simulink model "PreCondition"  (R2018b)
settings: Solver=FixedStepDiscrete  StartTime=0.0  StopTime=10.0  FixedStep=0.01  RelTol=1e-3
undefined symbols (not defined in the file or in its folder): EnergyMgLdShdRq1, HMI_2L_StMd10_Config_Val, HMI_2L_StMd11_Config_Val, HMI_2L_StMd12_Config_Val, HMI_2L_StMd13_Config_Val, HMI_2L_StMd14_Config_Val, HMI_2L_StMd15_Config_Val, HMI_2L_StMd16_Config_Val, HMI_2L_StMd17_Config_Val, HMI_2L_StMd18_Config_Val, HMI_2L_StMd19_Config_Val, HMI_2L_StMd1_Config_Val, HMI_2L_StMd20_Config_Val, HMI_2L_StMd21_Config_Val, HMI_2L_StMd22_Config_Val, HMI_2L_StMd23_Config_Val, HMI_2L_StMd24_Config_Val, HMI_2L_StMd25_Config_Val, HMI_2L_StMd26_Config_Val, HMI_2L_StMd27_Config_Val, HMI_2L_StMd28_Config_Val, HMI_2L_StMd29_Config_Val, HMI_2L_StMd2_Config_Val, HMI_2L_StMd30_Config_Val, HMI_2L_StMd31_Config_Val, HMI_2L_StMd32_Config_Val, HMI_2L_StMd3_Config_Val, HMI_2L_StMd4_Config_Val, HMI_2L_StMd5_Config_Val, HMI_2L_StMd6_Config_Val, HMI_2L_StMd7_Config_Val, HMI_2L_StMd8_Config_Val, HMI_2L_StMd9_Config_Val, HMI_2R_StMd10_Config_Val, HMI_2R_StMd11_Config_Val, HMI_2R_StMd12_Config_Val, HMI_2R_StMd13_Config_Val, HMI_2R_StMd14_Config_Val, HMI_2R_StMd15_Config_Val, HMI_2R_StMd16_Config_Val, HMI_2R_StMd17_Config_Val, HMI_2R_StMd18_Config_Val, HMI_2R_StMd19_Config_Val, HMI_2R_StMd1_Config_Val, HMI_2R_StMd20_Config_Val, HMI_2R_StMd21_Config_Val, HMI_2R_StMd22_Config_Val, HMI_2R_StMd23_Config_Val, HMI_2R_StMd24_Config_Val, HMI_2R_StMd25_Config_Val, HMI_2R_StMd26_Config_Val, HMI_2R_StMd27_Config_Val, HMI_2R_StMd28_Config_Val, HMI_2R_StMd29_Config_Val, HMI_2R_StMd2_Config_Val, HMI_2R_StMd30_Config_Val, HMI_2R_StMd31_Config_Val, HMI_2R_StMd32_Config_Val, HMI_2R_StMd3_Config_Val, HMI_2R_StMd4_Config_Val ... (+94)
(part 1 of 6)
settings Model: PauseTimes=0.01  Creator=su3dcu  LastModifiedBy=su3dcu
settings DataIOCC: SaveFormat=StructureWithTime  ReturnWorkspaceOutputs=on
settings OptimizationCC: DefaultParameterBehavior=Inlined  EnhancedBackFolding=on  PassReuseOutputArgsAs=Individual arguments  ZeroExternalMemoryAtStartup=off  ZeroInternalMemoryAtStartup=off  OptimizeBlockOrder=speed  DifferentSizesBufferReuse=on  OptimizationCustomize=off
settings DebuggingCC: ParameterTunabilityLossMsg=error
settings HardwareCC: ProdBitPerPointer=32  ProdBitPerSizeT=32  ProdBitPerPtrDiffT=32  ProdLargestAtomicFloat=None  ProdWordSize=32  ProdHWDeviceType=Renesas->RH850
settings ModelReferenceCC: ModelReferenceNumInstancesAllowed=Single
settings SFSimCC: SimCustomHeaderCode="#include\"Rte_Type.h\""  MATLABDynamicMemAlloc=off
settings RTWCC: SystemTargetFile=autosar.tlc  GenCodeOnly=on  TemplateMakefile=ert_default_tmf  Description=AUTOSAR  GenerateReport=on  IncludeHyperlinkInReport=on  LaunchReport=on  CodeExecutionProfiling=on  GenerateTraceInfo=on  GenerateTraceReport=on  GenerateTraceReportSl=on  GenerateTraceReportSf=on  GenerateTraceReportEml=on  GenerateCodeMetricsReport=on
settings CodeAppCC: ForceParamTrailComments=on  IgnoreCustomStorageClasses=off  MaxIdLength=63  OperatorAnnotations=on  SimulinkDataObjDesc=on  SFDataObjDesc=on  InsertBlockDesc=on
settings STFCustomTargetCC: TargetLangStandard=C99 (ISO)  MultiwordLength=256  ParMdlRefBuildCompliant=on  CompOptLevelCompliant=on  IncludeMdlTerminateFcn=off  CombineOutputUpdateFcns=on  SuppressErrorStatus=on  ERTCustomFileBanners=on  SupportAbsoluteTime=off  PurelyIntegerCode=on  SupportNonFinite=off  SupportComplex=off  SupportContinuousTime=off  SupportNonInlinedSFcns=off  RemoveResetFunc=on  MATLABClassNameForMDSCustomization=Simulink.SoftwareTarget.ERTCustomization  AutosarCompliant=on  UseToolchainInfoCompliant=on  LookupTableObjectStructAxisOrder=2,1,3,4,...  LUTObjectStructOrderEvenSpacing=Size,Table,Breakpoints  SystemTargetFile=autosar.tlc
settings ERTTargetCC: TargetLangStandard=C99 (ISO)  ConcurrentExecutionCompliant=off  IncludeMdlTerminateFcn=off  SuppressErrorStatus=on  SupportAbsoluteTime=off  PurelyIntegerCode=on  SupportNonFinite=off  SupportComplex=off  ModelStepFunctionPrototypeControlCompliant=off  CPPClassGenCompliant=off  AutosarCompliant=on  LookupTableObjectStructAxisOrder=2,1,3,4,...  LUTObjectStructOrderEvenSpacing=Size,Table,Breakpoints  InlinedParameterPlacement=NonHierarchical  ERTCustomFileTemplate=example_file_process.tlc  ERTFilePackagingFormat=Compact
settings ConfigComp: DVTestSuiteOptimization=CombinedObjectives (Nonlinear Extended)  DVDetectActiveLogic=on  DVDetectOutOfBounds=on

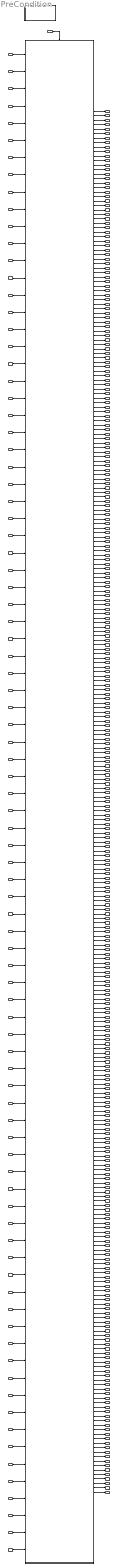
== system PreCondition ==
  PreConitionRunnable : Inport  SampleTime=0.01  OutputFunctionCall=on
  AbgDplyBckp_Val : Inport  Port=2  OutDataTypeStr=boolean  PortDimensions=1
  AbgDplyBckpV_Val : Inport  Port=3  OutDataTypeStr=boolean  PortDimensions=1
  AcsEntryPosLrnd_Val : Inport  Port=4  OutDataTypeStr=PosLrnd1  PortDimensions=1
  DrvStPosRclRspStat_Val : Inport  Port=5  OutDataTypeStr=Enum: PosRclRspStat1  PortDimensions=1
  EnergyMgLdShdRq_Val : Inport  Port=6  OutDataTypeStr=Enum: EnergyMgLdShdRq1  PortDimensions=1
  FamilyLtPosLrnd_Val : Inport  Port=7  OutDataTypeStr=PosLrnd1  PortDimensions=1
  FamilyRtPosLrnd_Val : Inport  Port=8  OutDataTypeStr=PosLrnd1  PortDimensions=1
  IfVeSMSeStNumConfig_Val : Inport  Port=9  OutDataTypeStr=Enum: IfVeSMSeStNumConfig  PortDimensions=1
  IntimacyLPosLrnd_Val : Inport  Port=10  OutDataTypeStr=PosLrnd1  PortDimensions=1
  IntimacyRPosLrnd_Val : Inport  Port=11  OutDataTypeStr=PosLrnd1  PortDimensions=1
  Is2LStSwAct_Val : Inport  Port=12  OutDataTypeStr=boolean  PortDimensions=1
  Is2RStSwAct_Val : Inport  Port=13  OutDataTypeStr=boolean  PortDimensions=1
  Is3LStSwAct_Val : Inport  Port=14  OutDataTypeStr=boolean  PortDimensions=1
  Is3RStSwAct_Val : Inport  Port=15  OutDataTypeStr=boolean  PortDimensions=1
  IsDrvStSwAct_Val : Inport  Port=16  OutDataTypeStr=boolean  PortDimensions=1
  IsPasStSwAct_Val : Inport  Port=17  OutDataTypeStr=boolean  PortDimensions=1
  LgrstCloseLtPosLrnd_Val : Inport  Port=18  OutDataTypeStr=PosLrnd1  PortDimensions=1
  LgrstCloseRtPosLrnd_Val : Inport  Port=19  OutDataTypeStr=PosLrnd1  PortDimensions=1
  LgrstOpenLtPosLrnd_Val : Inport  Port=20  OutDataTypeStr=PosLrnd1  PortDimensions=1
  LgrstOpenRtPosLrnd_Val : Inport  Port=21  OutDataTypeStr=PosLrnd1  PortDimensions=1
  LugLtPosLrnd_Val : Inport  Port=22  OutDataTypeStr=PosLrnd1  PortDimensions=1
  LugRtPosLrnd_Val : Inport  Port=23  OutDataTypeStr=PosLrnd1  PortDimensions=1
  LyingLtPosLrnd_Val : Inport  Port=24  OutDataTypeStr=PosLrnd1  PortDimensions=1
  LyingRtPosLrnd_Val : Inport  Port=25  OutDataTypeStr=PosLrnd1  PortDimensions=1
  MmryRclImpctDisRq_Val : Inport  Port=26  OutDataTypeStr=uint8  PortDimensions=1
  AcsExitPosLrnd_Val : Inport  Port=27  OutDataTypeStr=PosLrnd1  PortDimensions=1
  PassStPosRclRspStat_Val : Inport  Port=28  OutDataTypeStr=Enum: PosRclRspStat1  PortDimensions=1
  VIPLtPosLrnd_Val : Inport  Port=29  OutDataTypeStr=PosLrnd1  PortDimensions=1
  SecRwLtStChldLkReq_Val : Inport  Port=30  OutDataTypeStr=Enum: SeatChldLkSt  PortDimensions=1
  SecRwLtStPosRclRspStat_Val : Inport  Port=31  OutDataTypeStr=Enum: PosRclRspStat1  PortDimensions=1
  VIPRtPosLrnd_Val : Inport  Port=32  OutDataTypeStr=PosLrnd1  PortDimensions=1
  SecRwRtStChldLkReq_Val : Inport  Port=33  OutDataTypeStr=Enum: SeatChldLkSt  PortDimensions=1
  SecRwRtStPosRclRspStat_Val : Inport  Port=34  OutDataTypeStr=Enum: PosRclRspStat1  PortDimensions=1
  SysPwrMd_Val : Inport  Port=35  OutDataTypeStr=Enum: PowerMode1  PortDimensions=1
  SysPwrMdV_Val : Inport  Port=36  OutDataTypeStr=boolean  PortDimensions=1
  ThdRwCtStOccStatMSMSrc_Val : Inport  Port=37  OutDataTypeStr=Enum: SeatOccupiedSts1  PortDimensions=1
  RcvyLtPosLrnd_Val : Inport  Port=38  OutDataTypeStr=PosLrnd1  PortDimensions=1
  ThdRwLtStOccStatMSMSrc_Val : Inport  Port=39  OutDataTypeStr=Enum: SeatOccupiedSts1  PortDimensions=1
  ThdRwLtStPosRclRspStat_Val : Inport  Port=40  OutDataTypeStr=Enum: PosRclRspStat1  PortDimensions=1
  RcvyRtPosLrnd_Val : Inport  Port=41  OutDataTypeStr=PosLrnd1  PortDimensions=1
  ThdRwRtStOccStatMSMSrc_Val : Inport  Port=42  OutDataTypeStr=Enum: SeatOccupiedSts1  PortDimensions=1
  ThdRwRtStPosRclRspStat_Val : Inport  Port=43  OutDataTypeStr=Enum: PosRclRspStat1  PortDimensions=1
  VehMovState_Val : Inport  Port=44  OutDataTypeStr=Enum: VehMovState1  PortDimensions=1
  VehSpdAvgDrvn_Val : Inport  Port=45  OutDataTypeStr=uint16  PortDimensions=1
  VehSpdAvgDrvnV_Val : Inport  Port=46  OutDataTypeStr=boolean  PortDimensions=1
  VeSignalLost2R_463_2L_Val : Inport  Port=47  OutDataTypeStr=boolean  PortDimensions=1
  VeSignalLost3L_468_2L_Val : Inport  Port=48  OutDataTypeStr=boolean  PortDimensions=1
  VeSignalLost3R_46C_2L_Val : Inport  Port=49  OutDataTypeStr=boolean  PortDimensions=1
  VeSignalLostCODR_470_2L_Val : Inport  Port=50  OutDataTypeStr=boolean  PortDimensions=1
  VeSignalLostDR_213_2L_Val : Inport  Port=51  OutDataTypeStr=boolean  PortDimensions=1
  VeSignalLostFireWall_1D2_2L_Val : Inport  Port=52  OutDataTypeStr=boolean  PortDimensions=1
  VeSignalLostSDM_195_2L_Val : Inport  Port=53  OutDataTypeStr=boolean  PortDimensions=1
  VoltSts_Val : Inport  Port=54  OutDataTypeStr=Enum: SeatSysVoltSt  PortDimensions=1
  SecRwLtStFrwdBkwdPos_Val : Inport  Port=55  OutDataTypeStr=uint16  PortDimensions=1
  SecRwLtStFrwdBkwdPosV_Val : Inport  Port=56  OutDataTypeStr=boolean  PortDimensions=1
  SecRwRtStFrwdBkwdPos_Val : Inport  Port=57  OutDataTypeStr=uint16  PortDimensions=1
  SecRwRtStFrwdBkwdPosV_Val : Inport  Port=58  OutDataTypeStr=boolean  PortDimensions=1
  AcsEntry4s2LPosLrnd_Val : Inport  Port=59  OutDataTypeStr=PosLrnd1  PortDimensions=1
  AcsEntry4s2RPosLrnd_Val : Inport  Port=60  OutDataTypeStr=PosLrnd1  PortDimensions=1
  AcsEntryAll4sBwdPosLrnd_Val : Inport  Port=61  OutDataTypeStr=PosLrnd1  PortDimensions=1
  AcsEntryAll4sFwdPosLrnd_Val : Inport  Port=62  OutDataTypeStr=PosLrnd1  PortDimensions=1
  AcsExit4s2LPosLrnd_Val : Inport  Port=63  OutDataTypeStr=PosLrnd1  PortDimensions=1
  AcsExit4s2RPosLrnd_Val : Inport  Port=64  OutDataTypeStr=PosLrnd1  PortDimensions=1
  IfVeSMSbPassReclinerPosLrnd_Val : Inport  Port=65  OutDataTypeStr=PosLrnd1  PortDimensions=1
  IfVeSMSbunfold3LPosLrnd_Val : Inport  Port=66  OutDataTypeStr=PosLrnd1  PortDimensions=1
  IfVeSMSbunfold3RPosLrnd_Val : Inport  Port=67  OutDataTypeStr=PosLrnd1  PortDimensions=1
  NotCoDrvStOccStatBDFSrc_Val : Inport  Port=68  OutDataTypeStr=Enum: SeatOccupiedSts1  PortDimensions=1
  IfVeSMSbVIPLtOutPosLrnd_Val : Inport  Port=69  OutDataTypeStr=PosLrnd1  PortDimensions=1
  IfVeSMSbVIPRtOutPosLrnd_Val : Inport  Port=70  OutDataTypeStr=PosLrnd1  PortDimensions=1
  IfVeSMSuThdRwLtStCshnFldUpwdDnwdPos_Val : Inport  Port=71  OutDataTypeStr=uint16  PortDimensions=1
  IfVeSMSuThdRwLtStCshnFldUpwdDnwdPosV_Val : Inport  Port=72  OutDataTypeStr=boolean  PortDimensions=1
  IfVeSMSuThdRwRtStCshnFldUpwdDnwdPos_Val : Inport  Port=73  OutDataTypeStr=uint16  PortDimensions=1
  IfVeSMSuThdRwRtStCshnFldUpwdDnwdPosV_Val : Inport  Port=74  OutDataTypeStr=boolean  PortDimensions=1
  ThdRwLtStChldLkReq_Val : Inport  Port=75  OutDataTypeStr=Enum: SeatChldLkSt  PortDimensions=1
  NotSecRowLeStOccStatBDFSrc_Val : Inport  Port=76  OutDataTypeStr=Enum: SeatOccupiedSts1  PortDimensions=1
  NotSecRowRtStOccStatBDFSrc_Val : Inport  Port=77  OutDataTypeStr=Enum: SeatOccupiedSts1  PortDimensions=1
  IfVeSMSbSecRwLtStBkReclnUpwdDnwdPosV_Val : Inport  Port=78  OutDataTypeStr=boolean  PortDimensions=1
  IfVeSMSbSecRwRtStBkReclnUpwdDnwdPosV_Val : Inport  Port=79  OutDataTypeStr=boolean  PortDimensions=1
  IfVeSMSuSecRwLtStBkReclnUpwdDnwdPos_Val : Inport  Port=80  OutDataTypeStr=uint16  PortDimensions=1
  IfVeSMSuSecRwRtStBkReclnUpwdDnwdPos_Val : Inport  Port=81  OutDataTypeStr=uint16  PortDimensions=1
  IfVeSMSbPasReclinerPosAvail_Val : Inport  Port=82  OutDataTypeStr=boolean  PortDimensions=1
  WholeVehMemPosLrnd_Val : Inport  Port=83  OutDataTypeStr=PosLrnd1  PortDimensions=1
  Md61PassStBkReclnTrgtPos_Val : Inport  Port=84  OutDataTypeStr=uint16  PortDimensions=1
  Md61ThdRwLtStCshnFldUpwdDnwdTrgtPos_Val : Inport  Port=85  OutDataTypeStr=uint16  PortDimensions=1
  Md61ThdRwRtStCshnFldUpwdDnwdTrgtPos_Val : Inport  Port=86  OutDataTypeStr=uint16  PortDimensions=1
  Md62PassStBkReclnTrgtPos_Val : Inport  Port=87  OutDataTypeStr=uint16  PortDimensions=1
  Md62ThdRwLtStCshnFldUpwdDnwdTrgtPos_Val : Inport  Port=88  OutDataTypeStr=uint16  PortDimensions=1
  Md62ThdRwRtStCshnFldUpwdDnwdTrgtPos_Val : Inport  Port=89  OutDataTypeStr=uint16  PortDimensions=1
  PreCondition_Init : Subsystem
  PreConitionRunnable_sys : Subsystem
  AcsMdEntyAvl_Val : Outport  OutDataTypeStr=boolean  PortDimensions=1
  AcsMdExtAvl_Val : Outport  Port=2  OutDataTypeStr=boolean  PortDimensions=1
  CommCond_Val : Outport  Port=3  OutDataTypeStr=boolean  PortDimensions=1
  CommExitCond_Val : Outport  Port=4  OutDataTypeStr=boolean  PortDimensions=1
  CommExitCondwithSpeed_Val : Outport  Port=5  OutDataTypeStr=boolean  PortDimensions=1
  DiagAbgDly_Val : Outport  Port=6  OutDataTypeStr=Enum: DiagAbgDly  PortDimensions=1
  DiagVehMovState_Val : Outport  Port=7  OutDataTypeStr=Enum: DiagVehMovState  PortDimensions=1
  DiagVehSpdAvgDrvn_Val : Outport  Port=8  OutDataTypeStr=Enum: DiagVehSpdAvgDrvn  PortDimensions=1
  FamilyMdLtAvl_Val : Outport  Port=9  OutDataTypeStr=boolean  PortDimensions=1
  FamilyMdRtAvl_Val : Outport  Port=10  OutDataTypeStr=boolean  PortDimensions=1
  HMIMd10Avl_2L_Val : Outport  Port=11  OutDataTypeStr=boolean  PortDimensions=1
  HMIMd10Avl_2R_Val : Outport  Port=12  OutDataTypeStr=boolean  PortDimensions=1
  HMIMd10Cfg_2L_Val : Outport  Port=13  OutDataTypeStr=boolean  PortDimensions=1
  HMIMd10Cfg_2R_Val : Outport  Port=14  OutDataTypeStr=boolean  PortDimensions=1
  HMIMd11Avl_2L_Val : Outport  Port=15  OutDataTypeStr=boolean  PortDimensions=1
  HMIMd11Avl_2R_Val : Outport  Port=16  OutDataTypeStr=boolean  PortDimensions=1
  HMIMd11Cfg_2L_Val : Outport  Port=17  OutDataTypeStr=boolean  PortDimensions=1
  HMIMd11Cfg_2R_Val : Outport  Port=18  OutDataTypeStr=boolean  PortDimensions=1
  HMIMd12Avl_2L_Val : Outport  Port=19  OutDataTypeStr=boolean  PortDimensions=1
  HMIMd12Avl_2R_Val : Outport  Port=20  OutDataTypeStr=boolean  PortDimensions=1
  HMIMd12Cfg_2L_Val : Outport  Port=21  OutDataTypeStr=boolean  PortDimensions=1
  HMIMd12Cfg_2R_Val : Outport  Port=22  OutDataTypeStr=boolean  PortDimensions=1
  HMIMd13Avl_2L_Val : Outport  Port=23  OutDataTypeStr=boolean  PortDimensions=1
  HMIMd13Avl_2R_Val : Outport  Port=24  OutDataTypeStr=boolean  PortDimensions=1
  HMIMd13Cfg_2L_Val : Outport  Port=25  OutDataTypeStr=boolean  PortDimensions=1
  HMIMd13Cfg_2R_Val : Outport  Port=26  OutDataTypeStr=boolean  PortDimensions=1
  HMIMd14Avl_2L_Val : Outport  Port=27  OutDataTypeStr=boolean  PortDimensions=1
  HMIMd14Avl_2R_Val : Outport  Port=28  OutDataTypeStr=boolean  PortDimensions=1
  HMIMd14Cfg_2L_Val : Outport  Port=29  OutDataTypeStr=boolean  PortDimensions=1
  HMIMd14Cfg_2R_Val : Outport  Port=30  OutDataTypeStr=boolean  PortDimensions=1
  HMIMd15Avl_2L_Val : Outport  Port=31  OutDataTypeStr=boolean  PortDimensions=1
  HMIMd15Avl_2R_Val : Outport  Port=32  OutDataTypeStr=boolean  PortDimensions=1
  HMIMd15Cfg_2L_Val : Outport  Port=33  OutDataTypeStr=boolean  PortDimensions=1
  HMIMd15Cfg_2R_Val : Outport  Port=34  OutDataTypeStr=boolean  PortDimensions=1
  HMIMd16Avl_2L_Val : Outport  Port=35  OutDataTypeStr=boolean  PortDimensions=1
  HMIMd16Avl_2R_Val : Outport  Port=36  OutDataTypeStr=boolean  PortDimensions=1
  HMIMd16Cfg_2L_Val : Outport  Port=37  OutDataTypeStr=boolean  PortDimensions=1
  HMIMd16Cfg_2R_Val : Outport  Port=38  OutDataTypeStr=boolean  PortDimensions=1
  HMIMd17Avl_2L_Val : Outport  Port=39  OutDataTypeStr=boolean  PortDimensions=1
  HMIMd17Avl_2R_Val : Outport  Port=40  OutDataTypeStr=boolean  PortDimensions=1
  HMIMd17Cfg_2L_Val : Outport  Port=41  OutDataTypeStr=boolean  PortDimensions=1
  HMIMd17Cfg_2R_Val : Outport  Port=42  OutDataTypeStr=boolean  PortDimensions=1
  HMIMd18Avl_2L_Val : Outport  Port=43  OutDataTypeStr=boolean  PortDimensions=1
  HMIMd18Avl_2R_Val : Outport  Port=44  OutDataTypeStr=boolean  PortDimensions=1
  HMIMd18Cfg_2L_Val : Outport  Port=45  OutDataTypeStr=boolean  PortDimensions=1
  HMIMd18Cfg_2R_Val : Outport  Port=46  OutDataTypeStr=boolean  PortDimensions=1
  HMIMd19Avl_2L_Val : Outport  Port=47  OutDataTypeStr=boolean  PortDimensions=1
  HMIMd19Avl_2R_Val : Outport  Port=48  OutDataTypeStr=boolean  PortDimensions=1
  HMIMd19Cfg_2L_Val : Outport  Port=49  OutDataTypeStr=boolean  PortDimensions=1
  HMIMd19Cfg_2R_Val : Outport  Port=50  OutDataTypeStr=boolean  PortDimensions=1
  HMIMd1Avl_2L_Val : Outport  Port=51  OutDataTypeStr=boolean  PortDimensions=1
  HMIMd1Avl_2R_Val : Outport  Port=52  OutDataTypeStr=boolean  PortDimensions=1
  HMIMd1Cfg_2L_Val : Outport  Port=53  OutDataTypeStr=boolean  PortDimensions=1
  HMIMd1Cfg_2R_Val : Outport  Port=54  OutDataTypeStr=boolean  PortDimensions=1
  HMIMd20Avl_2L_Val : Outport  Port=55  OutDataTypeStr=boolean  PortDimensions=1
  HMIMd20Avl_2R_Val : Outport  Port=56  OutDataTypeStr=boolean  PortDimensions=1
  HMIMd20Cfg_2L_Val : Outport  Port=57  OutDataTypeStr=boolean  PortDimensions=1
  HMIMd20Cfg_2R_Val : Outport  Port=58  OutDataTypeStr=boolean  PortDimensions=1
  HMIMd21Avl_2L_Val : Outport  Port=59  OutDataTypeStr=boolean  PortDimensions=1
  HMIMd21Avl_2R_Val : Outport  Port=60  OutDataTypeStr=boolean  PortDimensions=1
  HMIMd21Cfg_2L_Val : Outport  Port=61  OutDataTypeStr=boolean  PortDimensions=1
  HMIMd21Cfg_2R_Val : Outport  Port=62  OutDataTypeStr=boolean  PortDimensions=1
  HMIMd22Avl_2L_Val : Outport  Port=63  OutDataTypeStr=boolean  PortDimensions=1
  HMIMd22Avl_2R_Val : Outport  Port=64  OutDataTypeStr=boolean  PortDimensions=1
  HMIMd22Cfg_2L_Val : Outport  Port=65  OutDataTypeStr=boolean  PortDimensions=1
  HMIMd22Cfg_2R_Val : Outport  Port=66  OutDataTypeStr=boolean  PortDimensions=1
  HMIMd23Avl_2L_Val : Outport  Port=67  OutDataTypeStr=boolean  PortDimensions=1
  HMIMd23Avl_2R_Val : Outport  Port=68  OutDataTypeStr=boolean  PortDimensions=1
  HMIMd23Cfg_2L_Val : Outport  Port=69  OutDataTypeStr=boolean  PortDimensions=1
  HMIMd23Cfg_2R_Val : Outport  Port=70  OutDataTypeStr=boolean  PortDimensions=1
  HMIMd24Avl_2L_Val : Outport  Port=71  OutDataTypeStr=boolean  PortDimensions=1
  HMIMd24Avl_2R_Val : Outport  Port=72  OutDataTypeStr=boolean  PortDimensions=1
  HMIMd24Cfg_2L_Val : Outport  Port=73  OutDataTypeStr=boolean  PortDimensions=1
  HMIMd24Cfg_2R_Val : Outport  Port=74  OutDataTypeStr=boolean  PortDimensions=1
  HMIMd25Avl_2L_Val : Outport  Port=75  OutDataTypeStr=boolean  PortDimensions=1
  HMIMd25Avl_2R_Val : Outport  Port=76  OutDataTypeStr=boolean  PortDimensions=1
  HMIMd25Cfg_2L_Val : Outport  Port=77  OutDataTypeStr=boolean  PortDimensions=1
  HMIMd25Cfg_2R_Val : Outport  Port=78  OutDataTypeStr=boolean  PortDimensions=1
  HMIMd26Avl_2L_Val : Outport  Port=79  OutDataTypeStr=boolean  PortDimensions=1
  HMIMd26Avl_2R_Val : Outport  Port=80  OutDataTypeStr=boolean  PortDimensions=1
  HMIMd26Cfg_2L_Val : Outport  Port=81  OutDataTypeStr=boolean  PortDimensions=1
  HMIMd26Cfg_2R_Val : Outport  Port=82  OutDataTypeStr=boolean  PortDimensions=1
  HMIMd27Avl_2L_Val : Outport  Port=83  OutDataTypeStr=boolean  PortDimensions=1
  HMIMd27Avl_2R_Val : Outport  Port=84  OutDataTypeStr=boolean  PortDimensions=1
  HMIMd27Cfg_2L_Val : Outport  Port=85  OutDataTypeStr=boolean  PortDimensions=1
  HMIMd27Cfg_2R_Val : Outport  Port=86  OutDataTypeStr=boolean  PortDimensions=1
  HMIMd28Avl_2L_Val : Outport  Port=87  OutDataTypeStr=boolean  PortDimensions=1
  HMIMd28Avl_2R_Val : Outport  Port=88  OutDataTypeStr=boolean  PortDimensions=1
  HMIMd28Cfg_2L_Val : Outport  Port=89  OutDataTypeStr=boolean  PortDimensions=1
  HMIMd28Cfg_2R_Val : Outport  Port=90  OutDataTypeStr=boolean  PortDimensions=1
  HMIMd29Avl_2L_Val : Outport  Port=91  OutDataTypeStr=boolean  PortDimensions=1
  HMIMd29Avl_2R_Val : Outport  Port=92  OutDataTypeStr=boolean  PortDimensions=1
  HMIMd29Cfg_2L_Val : Outport  Port=93  OutDataTypeStr=boolean  PortDimensions=1
  HMIMd29Cfg_2R_Val : Outport  Port=94  OutDataTypeStr=boolean  PortDimensions=1
  HMIMd2Avl_2L_Val : Outport  Port=95  OutDataTypeStr=boolean  PortDimensions=1
  HMIMd2Avl_2R_Val : Outport  Port=96  OutDataTypeStr=boolean  PortDimensions=1
  HMIMd2Cfg_2L_Val : Outport  Port=97  OutDataTypeStr=boolean  PortDimensions=1
  HMIMd2Cfg_2R_Val : Outport  Port=98  OutDataTypeStr=boolean  PortDimensions=1
  HMIMd30Avl_2L_Val : Outport  Port=99  OutDataTypeStr=boolean  PortDimensions=1
  HMIMd30Avl_2R_Val : Outport  Port=100  OutDataTypeStr=boolean  PortDimensions=1
  HMIMd30Cfg_2L_Val : Outport  Port=101  OutDataTypeStr=boolean  PortDimensions=1
  HMIMd30Cfg_2R_Val : Outport  Port=102  OutDataTypeStr=boolean  PortDimensions=1
  HMIMd31Avl_2L_Val : Outport  Port=103  OutDataTypeStr=boolean  PortDimensions=1
  HMIMd31Avl_2R_Val : Outport  Port=104  OutDataTypeStr=boolean  PortDimensions=1
  HMIMd31Cfg_2L_Val : Outport  Port=105  OutDataTypeStr=boolean  PortDimensions=1
  HMIMd31Cfg_2R_Val : Outport  Port=106  OutDataTypeStr=boolean  PortDimensions=1
  HMIMd32Avl_2L_Val : Outport  Port=107  OutDataTypeStr=boolean  PortDimensions=1
  HMIMd32Avl_2R_Val : Outport  Port=108  OutDataTypeStr=boolean  PortDimensions=1
  HMIMd32Cfg_2L_Val : Outport  Port=109  OutDataTypeStr=boolean  PortDimensions=1
  HMIMd32Cfg_2R_Val : Outport  Port=110  OutDataTypeStr=boolean  PortDimensions=1
  HMIMd3Avl_2L_Val : Outport  Port=111  OutDataTypeStr=boolean  PortDimensions=1
  HMIMd3Avl_2R_Val : Outport  Port=112  OutDataTypeStr=boolean  PortDimensions=1
  HMIMd3Cfg_2L_Val : Outport  Port=113  OutDataTypeStr=boolean  PortDimensions=1
  HMIMd3Cfg_2R_Val : Outport  Port=114  OutDataTypeStr=boolean  PortDimensions=1
  HMIMd4Avl_2L_Val : Outport  Port=115  OutDataTypeStr=boolean  PortDimensions=1
  HMIMd4Avl_2R_Val : Outport  Port=116  OutDataTypeStr=boolean  PortDimensions=1
  HMIMd4Cfg_2L_Val : Outport  Port=117  OutDataTypeStr=boolean  PortDimensions=1
  HMIMd4Cfg_2R_Val : Outport  Port=118  OutDataTypeStr=boolean  PortDimensions=1
  HMIMd5Avl_2L_Val : Outport  Port=119  OutDataTypeStr=boolean  PortDimensions=1
  HMIMd5Avl_2R_Val : Outport  Port=120  OutDataTypeStr=boolean  PortDimensions=1
  HMIMd5Cfg_2L_Val : Outport  Port=121  OutDataTypeStr=boolean  PortDimensions=1
  HMIMd5Cfg_2R_Val : Outport  Port=122  OutDataTypeStr=boolean  PortDimensions=1
  HMIMd6Avl_2L_Val : Outport  Port=123  OutDataTypeStr=boolean  PortDimensions=1
  HMIMd6Avl_2R_Val : Outport  Port=124  OutDataTypeStr=boolean  PortDimensions=1
  HMIMd6Cfg_2L_Val : Outport  Port=125  OutDataTypeStr=boolean  PortDimensions=1
  HMIMd6Cfg_2R_Val : Outport  Port=126  OutDataTypeStr=boolean  PortDimensions=1
  HMIMd7Avl_2L_Val : Outport  Port=127  OutDataTypeStr=boolean  PortDimensions=1
  HMIMd7Avl_2R_Val : Outport  Port=128  OutDataTypeStr=boolean  PortDimensions=1
  HMIMd7Cfg_2L_Val : Outport  Port=129  OutDataTypeStr=boolean  PortDimensions=1
  HMIMd7Cfg_2R_Val : Outport  Port=130  OutDataTypeStr=boolean  PortDimensions=1
  HMIMd8Avl_2L_Val : Outport  Port=131  OutDataTypeStr=boolean  PortDimensions=1
  HMIMd8Avl_2R_Val : Outport  Port=132  OutDataTypeStr=boolean  PortDimensions=1
  HMIMd8Cfg_2L_Val : Outport  Port=133  OutDataTypeStr=boolean  PortDimensions=1
  HMIMd8Cfg_2R_Val : Outport  Port=134  OutDataTypeStr=boolean  PortDimensions=1
  HMIMd9Avl_2L_Val : Outport  Port=135  OutDataTypeStr=boolean  PortDimensions=1
  HMIMd9Avl_2R_Val : Outport  Port=136  OutDataTypeStr=boolean  PortDimensions=1
  HMIMd9Cfg_2L_Val : Outport  Port=137  OutDataTypeStr=boolean  PortDimensions=1
  HMIMd9Cfg_2R_Val : Outport  Port=138  OutDataTypeStr=boolean  PortDimensions=1
  IntimacyLMdAvl_Val : Outport  Port=139  OutDataTypeStr=boolean  PortDimensions=1
  IntimacyRMdAvl_Val : Outport  Port=140  OutDataTypeStr=boolean  PortDimensions=1
  LgrstCloseLtMdAvl_Val : Outport  Port=141  OutDataTypeStr=boolean  PortDimensions=1
  LgrstCloseRtMdAvl_Val : Outport  Port=142  OutDataTypeStr=boolean  PortDimensions=1
  LgrstOpenLtMdAvl_Val : Outport  Port=143  OutDataTypeStr=boolean  PortDimensions=1
  LgrstOpenRtMdAvl_Val : Outport  Port=144  OutDataTypeStr=boolean  PortDimensions=1
  LugMdLtAvl_Val : Outport  Port=145  OutDataTypeStr=boolean  PortDimensions=1
  LugMdRtAvl_Val : Outport  Port=146  OutDataTypeStr=boolean  PortDimensions=1
  LyingMdLtAvl_Val : Outport  Port=147  OutDataTypeStr=boolean  PortDimensions=1
  LyingMdRtAvl_Val : Outport  Port=148  OutDataTypeStr=boolean  PortDimensions=1
  PwrMdChked_Val : Outport  Port=149  OutDataTypeStr=Enum: PowerMode1  PortDimensions=1
  RcvyMdLtAvl_Val : Outport  Port=150  OutDataTypeStr=boolean  PortDimensions=1
  RcvyMdRtAvl_Val : Outport  Port=151  OutDataTypeStr=boolean  PortDimensions=1
  StPassCmprtMdCtrl_Md1_VCUAvl_Val : Outport  Port=152  OutDataTypeStr=boolean  PortDimensions=1
  StPassCmprtMdCtrl_Md1_VCUCfg_Val : Outport  Port=153  OutDataTypeStr=boolean  PortDimensions=1
  StPassCmprtMdCtrl_Md10_VCUAvl_Val : Outport  Port=154  OutDataTypeStr=boolean  PortDimensions=1
  StPassCmprtMdCtrl_Md10_VCUCfg_Val : Outport  Port=155  OutDataTypeStr=boolean  PortDimensions=1
  StPassCmprtMdCtrl_Md11_VCUAvl_Val : Outport  Port=156  OutDataTypeStr=boolean  PortDimensions=1
  StPassCmprtMdCtrl_Md11_VCUCfg_Val : Outport  Port=157  OutDataTypeStr=boolean  PortDimensions=1
  StPassCmprtMdCtrl_Md12_VCUAvl_Val : Outport  Port=158  OutDataTypeStr=boolean  PortDimensions=1
  StPassCmprtMdCtrl_Md12_VCUCfg_Val : Outport  Port=159  OutDataTypeStr=boolean  PortDimensions=1
  StPassCmprtMdCtrl_Md13_VCUAvl_Val : Outport  Port=160  OutDataTypeStr=boolean  PortDimensions=1
  StPassCmprtMdCtrl_Md13_VCUCfg_Val : Outport  Port=161  OutDataTypeStr=boolean  PortDimensions=1
  StPassCmprtMdCtrl_Md14_VCUAvl_Val : Outport  Port=162  OutDataTypeStr=boolean  PortDimensions=1
  StPassCmprtMdCtrl_Md14_VCUCfg_Val : Outport  Port=163  OutDataTypeStr=boolean  PortDimensions=1
  StPassCmprtMdCtrl_Md15_VCUAvl_Val : Outport  Port=164  OutDataTypeStr=boolean  PortDimensions=1
  StPassCmprtMdCtrl_Md15_VCUCfg_Val : Outport  Port=165  OutDataTypeStr=boolean  PortDimensions=1
  StPassCmprtMdCtrl_Md16_VCUAvl_Val : Outport  Port=166  OutDataTypeStr=boolean  PortDimensions=1
  StPassCmprtMdCtrl_Md16_VCUCfg_Val : Outport  Port=167  OutDataTypeStr=boolean  PortDimensions=1
  StPassCmprtMdCtrl_Md17_VCUAvl_Val : Outport  Port=168  OutDataTypeStr=boolean  PortDimensions=1
  StPassCmprtMdCtrl_Md17_VCUCfg_Val : Outport  Port=169  OutDataTypeStr=boolean  PortDimensions=1
  StPassCmprtMdCtrl_Md18_VCUAvl_Val : Outport  Port=170  OutDataTypeStr=boolean  PortDimensions=1
  StPassCmprtMdCtrl_Md18_VCUCfg_Val : Outport  Port=171  OutDataTypeStr=boolean  PortDimensions=1
  StPassCmprtMdCtrl_Md19_VCUAvl_Val : Outport  Port=172  OutDataTypeStr=boolean  PortDimensions=1
  StPassCmprtMdCtrl_Md19_VCUCfg_Val : Outport  Port=173  OutDataTypeStr=boolean  PortDimensions=1
  StPassCmprtMdCtrl_Md2_VCUAvl_Val : Outport  Port=174  OutDataTypeStr=boolean  PortDimensions=1
  StPassCmprtMdCtrl_Md2_VCUCfg_Val : Outport  Port=175  OutDataTypeStr=boolean  PortDimensions=1
  StPassCmprtMdCtrl_Md20_VCUAvl_Val : Outport  Port=176  OutDataTypeStr=boolean  PortDimensions=1
  StPassCmprtMdCtrl_Md20_VCUCfg_Val : Outport  Port=177  OutDataTypeStr=boolean  PortDimensions=1
  StPassCmprtMdCtrl_Md21_VCUAvl_Val : Outport  Port=178  OutDataTypeStr=boolean  PortDimensions=1
  StPassCmprtMdCtrl_Md21_VCUCfg_Val : Outport  Port=179  OutDataTypeStr=boolean  PortDimensions=1
  StPassCmprtMdCtrl_Md22_VCUAvl_Val : Outport  Port=180  OutDataTypeStr=boolean  PortDimensions=1
  StPassCmprtMdCtrl_Md22_VCUCfg_Val : Outport  Port=181  OutDataTypeStr=boolean  PortDimensions=1
  StPassCmprtMdCtrl_Md23_VCUAvl_Val : Outport  Port=182  OutDataTypeStr=boolean  PortDimensions=1
  StPassCmprtMdCtrl_Md23_VCUCfg_Val : Outport  Port=183  OutDataTypeStr=boolean  PortDimensions=1
  StPassCmprtMdCtrl_Md24_VCUAvl_Val : Outport  Port=184  OutDataTypeStr=boolean  PortDimensions=1
  StPassCmprtMdCtrl_Md24_VCUCfg_Val : Outport  Port=185  OutDataTypeStr=boolean  PortDimensions=1
  StPassCmprtMdCtrl_Md25_VCUAvl_Val : Outport  Port=186  OutDataTypeStr=boolean  PortDimensions=1
  StPassCmprtMdCtrl_Md25_VCUCfg_Val : Outport  Port=187  OutDataTypeStr=boolean  PortDimensions=1
  StPassCmprtMdCtrl_Md26_VCUAvl_Val : Outport  Port=188  OutDataTypeStr=boolean  PortDimensions=1
  StPassCmprtMdCtrl_Md26_VCUCfg_Val : Outport  Port=189  OutDataTypeStr=boolean  PortDimensions=1
  StPassCmprtMdCtrl_Md27_VCUAvl_Val : Outport  Port=190  OutDataTypeStr=boolean  PortDimensions=1
  StPassCmprtMdCtrl_Md27_VCUCfg_Val : Outport  Port=191  OutDataTypeStr=boolean  PortDimensions=1
  StPassCmprtMdCtrl_Md28_VCUAvl_Val : Outport  Port=192  OutDataTypeStr=boolean  PortDimensions=1
  StPassCmprtMdCtrl_Md28_VCUCfg_Val : Outport  Port=193  OutDataTypeStr=boolean  PortDimensions=1
  StPassCmprtMdCtrl_Md29_VCUAvl_Val : Outport  Port=194  OutDataTypeStr=boolean  PortDimensions=1
  StPassCmprtMdCtrl_Md29_VCUCfg_Val : Outport  Port=195  OutDataTypeStr=boolean  PortDimensions=1
  StPassCmprtMdCtrl_Md3_VCUAvl_Val : Outport  Port=196  OutDataTypeStr=boolean  PortDimensions=1
  StPassCmprtMdCtrl_Md3_VCUCfg_Val : Outport  Port=197  OutDataTypeStr=boolean  PortDimensions=1
  StPassCmprtMdCtrl_Md30_VCUAvl_Val : Outport  Port=198  OutDataTypeStr=boolean  PortDimensions=1
  StPassCmprtMdCtrl_Md30_VCUCfg_Val : Outport  Port=199  OutDataTypeStr=boolean  PortDimensions=1
  StPassCmprtMdCtrl_Md31_VCUAvl_Val : Outport  Port=200  OutDataTypeStr=boolean  PortDimensions=1
  StPassCmprtMdCtrl_Md31_VCUCfg_Val : Outport  Port=201  OutDataTypeStr=boolean  PortDimensions=1
  StPassCmprtMdCtrl_Md32_VCUAvl_Val : Outport  Port=202  OutDataTypeStr=boolean  PortDimensions=1
  StPassCmprtMdCtrl_Md32_VCUCfg_Val : Outport  Port=203  OutDataTypeStr=boolean  PortDimensions=1
  StPassCmprtMdCtrl_Md4_VCUAvl_Val : Outport  Port=204  OutDataTypeStr=boolean  PortDimensions=1
  StPassCmprtMdCtrl_Md4_VCUCfg_Val : Outport  Port=205  OutDataTypeStr=boolean  PortDimensions=1
  StPassCmprtMdCtrl_Md5_VCUAvl_Val : Outport  Port=206  OutDataTypeStr=boolean  PortDimensions=1
  StPassCmprtMdCtrl_Md5_VCUCfg_Val : Outport  Port=207  OutDataTypeStr=boolean  PortDimensions=1
  StPassCmprtMdCtrl_Md6_VCUAvl_Val : Outport  Port=208  OutDataTypeStr=boolean  PortDimensions=1
  StPassCmprtMdCtrl_Md6_VCUCfg_Val : Outport  Port=209  OutDataTypeStr=boolean  PortDimensions=1
  StPassCmprtMdCtrl_Md7_VCUAvl_Val : Outport  Port=210  OutDataTypeStr=boolean  PortDimensions=1
  StPassCmprtMdCtrl_Md7_VCUCfg_Val : Outport  Port=211  OutDataTypeStr=boolean  PortDimensions=1
  StPassCmprtMdCtrl_Md8_VCUAvl_Val : Outport  Port=212  OutDataTypeStr=boolean  PortDimensions=1
  StPassCmprtMdCtrl_Md8_VCUCfg_Val : Outport  Port=213  OutDataTypeStr=boolean  PortDimensions=1
  StPassCmprtMdCtrl_Md9_VCUAvl_Val : Outport  Port=214  OutDataTypeStr=boolean  PortDimensions=1
  StPassCmprtMdCtrl_Md9_VCUCfg_Val : Outport  Port=215  OutDataTypeStr=boolean  PortDimensions=1
  StPassCmprtMdRfCtrlSwCstStAvl_Val : Outport  Port=216  OutDataTypeStr=boolean  PortDimensions=1
  StSrvAvl_Md1_Val : Outport  Port=217  OutDataTypeStr=boolean  PortDimensions=1
  StSrvAvl_Md10_Val : Outport  Port=218  OutDataTypeStr=boolean  PortDimensions=1
  StSrvAvl_Md11_Val : Outport  Port=219  OutDataTypeStr=boolean  PortDimensions=1
  StSrvAvl_Md12_Val : Outport  Port=220  OutDataTypeStr=boolean  PortDimensions=1
  StSrvAvl_Md13_Val : Outport  Port=221  OutDataTypeStr=boolean  PortDimensions=1
  StSrvAvl_Md14_Val : Outport  Port=222  OutDataTypeStr=boolean  PortDimensions=1
  StSrvAvl_Md15_Val : Outport  Port=223  OutDataTypeStr=boolean  PortDimensions=1
  StSrvAvl_Md16_Val : Outport  Port=224  OutDataTypeStr=boolean  PortDimensions=1
  StSrvAvl_Md17_Val : Outport  Port=225  OutDataTypeStr=boolean  PortDimensions=1
  StSrvAvl_Md18_Val : Outport  Port=226  OutDataTypeStr=boolean  PortDimensions=1
  StSrvAvl_Md19_Val : Outport  Port=227  OutDataTypeStr=boolean  PortDimensions=1
  StSrvAvl_Md2_Val : Outport  Port=228  OutDataTypeStr=boolean  PortDimensions=1
  StSrvAvl_Md20_Val : Outport  Port=229  OutDataTypeStr=boolean  PortDimensions=1
  StSrvAvl_Md21_Val : Outport  Port=230  OutDataTypeStr=boolean  PortDimensions=1
  StSrvAvl_Md22_Val : Outport  Port=231  OutDataTypeStr=boolean  PortDimensions=1
  StSrvAvl_Md23_Val : Outport  Port=232  OutDataTypeStr=boolean  PortDimensions=1
  StSrvAvl_Md24_Val : Outport  Port=233  OutDataTypeStr=boolean  PortDimensions=1
  StSrvAvl_Md25_Val : Outport  Port=234  OutDataTypeStr=boolean  PortDimensions=1
  StSrvAvl_Md26_Val : Outport  Port=235  OutDataTypeStr=boolean  PortDimensions=1
  StSrvAvl_Md27_Val : Outport  Port=236  OutDataTypeStr=boolean  PortDimensions=1
  StSrvAvl_Md28_Val : Outport  Port=237  OutDataTypeStr=boolean  PortDimensions=1
  StSrvAvl_Md29_Val : Outport  Port=238  OutDataTypeStr=boolean  PortDimensions=1
  StSrvAvl_Md3_Val : Outport  Port=239  OutDataTypeStr=boolean  PortDimensions=1
  StSrvAvl_Md30_Val : Outport  Port=240  OutDataTypeStr=boolean  PortDimensions=1
  StSrvAvl_Md31_Val : Outport  Port=241  OutDataTypeStr=boolean  PortDimensions=1
  StSrvAvl_Md32_Val : Outport  Port=242  OutDataTypeStr=boolean  PortDimensions=1
  StSrvAvl_Md4_Val : Outport  Port=243  OutDataTypeStr=boolean  PortDimensions=1
  StSrvAvl_Md5_Val : Outport  Port=244  OutDataTypeStr=boolean  PortDimensions=1
  StSrvAvl_Md6_Val : Outport  Port=245  OutDataTypeStr=boolean  PortDimensions=1
  StSrvAvl_Md7_Val : Outport  Port=246  OutDataTypeStr=boolean  PortDimensions=1
  StSrvAvl_Md8_Val : Outport  Port=247  OutDataTypeStr=boolean  PortDimensions=1
  StSrvAvl_Md9_Val : Outport  Port=248  OutDataTypeStr=boolean  PortDimensions=1
  StSrvCfg_Md1_Val : Outport  Port=249  OutDataTypeStr=boolean  PortDimensions=1
  StSrvCfg_Md10_Val : Outport  Port=250  OutDataTypeStr=boolean  PortDimensions=1
  StSrvCfg_Md11_Val : Outport  Port=251  OutDataTypeStr=boolean  PortDimensions=1
  StSrvCfg_Md12_Val : Outport  Port=252  OutDataTypeStr=boolean  PortDimensions=1
  StSrvCfg_Md13_Val : Outport  Port=253  OutDataTypeStr=boolean  PortDimensions=1
  StSrvCfg_Md14_Val : Outport  Port=254  OutDataTypeStr=boolean  PortDimensions=1
  StSrvCfg_Md15_Val : Outport  Port=255  OutDataTypeStr=boolean  PortDimensions=1
  StSrvCfg_Md16_Val : Outport  Port=256  OutDataTypeStr=boolean  PortDimensions=1
  StSrvCfg_Md17_Val : Outport  Port=257  OutDataTypeStr=boolean  PortDimensions=1
  StSrvCfg_Md18_Val : Outport  Port=258  OutDataTypeStr=boolean  PortDimensions=1
  StSrvCfg_Md19_Val : Outport  Port=259  OutDataTypeStr=boolean  PortDimensions=1
  StSrvCfg_Md2_Val : Outport  Port=260  OutDataTypeStr=boolean  PortDimensions=1
  StSrvCfg_Md20_Val : Outport  Port=261  OutDataTypeStr=boolean  PortDimensions=1
  StSrvCfg_Md21_Val : Outport  Port=262  OutDataTypeStr=boolean  PortDimensions=1
  StSrvCfg_Md22_Val : Outport  Port=263  OutDataTypeStr=boolean  PortDimensions=1
  StSrvCfg_Md23_Val : Outport  Port=264  OutDataTypeStr=boolean  PortDimensions=1
  StSrvCfg_Md24_Val : Outport  Port=265  OutDataTypeStr=boolean  PortDimensions=1
  StSrvCfg_Md25_Val : Outport  Port=266  OutDataTypeStr=boolean  PortDimensions=1
  StSrvCfg_Md26_Val : Outport  Port=267  OutDataTypeStr=boolean  PortDimensions=1
  StSrvCfg_Md27_Val : Outport  Port=268  OutDataTypeStr=boolean  PortDimensions=1
  StSrvCfg_Md28_Val : Outport  Port=269  OutDataTypeStr=boolean  PortDimensions=1
  StSrvCfg_Md29_Val : Outport  Port=270  OutDataTypeStr=boolean  PortDimensions=1
  StSrvCfg_Md3_Val : Outport  Port=271  OutDataTypeStr=boolean  PortDimensions=1
  StSrvCfg_Md30_Val : Outport  Port=272  OutDataTypeStr=boolean  PortDimensions=1
  StSrvCfg_Md31_Val : Outport  Port=273  OutDataTypeStr=boolean  PortDimensions=1
  StSrvCfg_Md32_Val : Outport  Port=274  OutDataTypeStr=boolean  PortDimensions=1
  StSrvCfg_Md4_Val : Outport  Port=275  OutDataTypeStr=boolean  PortDimensions=1
  StSrvCfg_Md5_Val : Outport  Port=276  OutDataTypeStr=boolean  PortDimensions=1
  StSrvCfg_Md6_Val : Outport  Port=277  OutDataTypeStr=boolean  PortDimensions=1
  StSrvCfg_Md7_Val : Outport  Port=278  OutDataTypeStr=boolean  PortDimensions=1
  StSrvCfg_Md8_Val : Outport  Port=279  OutDataTypeStr=boolean  PortDimensions=1
  StSrvCfg_Md9_Val : Outport  Port=280  OutDataTypeStr=boolean  PortDimensions=1
  VipMdLtAvl_Val : Outport  Port=281  OutDataTypeStr=boolean  PortDimensions=1
  VipMdRtAvl_Val : Outport  Port=282  OutDataTypeStr=boolean  PortDimensions=1
  AcsEntry4s2LAvl_Val : Outport  Port=283  OutDataTypeStr=boolean  PortDimensions=1
  AcsEntry4s2RAvl_Val : Outport  Port=284  OutDataTypeStr=boolean  PortDimensions=1
  AcsEntryAll4sBwdAvl_Val : Outport  Port=285  OutDataTypeStr=boolean  PortDimensions=1
  AcsEntryAll4sFwdAvl_Val : Outport  Port=286  OutDataTypeStr=boolean  PortDimensions=1
  AcsExit4s2LAvl_Val : Outport  Port=287  OutDataTypeStr=boolean  PortDimensions=1
  AcsExit4s2RAvl_Val : Outport  Port=288  OutDataTypeStr=boolean  PortDimensions=1
  PasReclinerAvl_Val : Outport  Port=289  OutDataTypeStr=boolean  PortDimensions=1
  unfold3LAvl_Val : Outport  Port=290  OutDataTypeStr=boolean  PortDimensions=1
  unfold3RAvl_Val : Outport  Port=291  OutDataTypeStr=boolean  PortDimensions=1
  VipLtOutMdAvl_Val : Outport  Port=292  OutDataTypeStr=boolean  PortDimensions=1
  VipRtOutMdAvl_Val : Outport  Port=293  OutDataTypeStr=boolean  PortDimensions=1
  PasReclinerExitAvl_Val : Outport  Port=294  OutDataTypeStr=boolean  PortDimensions=1
  StPassCmprtMdCtrl_Md53_VCUAvl_Val : Outport  Port=295  OutDataTypeStr=boolean  PortDimensions=1
  StPassCmprtMdCtrl_Md53_VCUCfg_Val : Outport  Port=296  OutDataTypeStr=boolean  PortDimensions=1
  StPassCmprtMdCtrl_Md56_VCUAvl_Val : Outport  Port=297  OutDataTypeStr=boolean  PortDimensions=1
  StPassCmprtMdCtrl_Md56_VCUCfg_Val : Outport  Port=298  OutDataTypeStr=boolean  PortDimensions=1
  StPassCmprtMdCtrl_Md57_VCUAvl_Val : Outport  Port=299  OutDataTypeStr=boolean  PortDimensions=1
  StPassCmprtMdCtrl_Md57_VCUCfg_Val : Outport  Port=300  OutDataTypeStr=boolean  PortDimensions=1
  StPassCmprtMdCtrl_Md58_VCUAvl_Val : Outport  Port=301  OutDataTypeStr=boolean  PortDimensions=1
  StPassCmprtMdCtrl_Md58_VCUCfg_Val : Outport  Port=302  OutDataTypeStr=boolean  PortDimensions=1
  Big4SeatAvl_Val : Outport  Port=303  OutDataTypeStr=boolean  PortDimensions=1
  StPassCmprtMdCtrl_Md61_VCUAvl_Val : Outport  Port=304  OutDataTypeStr=boolean  PortDimensions=1
  StPassCmprtMdCtrl_Md62_VCUAvl_Val : Outport  Port=305  OutDataTypeStr=boolean  PortDimensions=1
  M61WholeVehMemAvl_Val : Outport  Port=306  OutDataTypeStr=boolean  PortDimensions=1
  M62WholeVehMemAvl_Val : Outport  Port=307  OutDataTypeStr=boolean  PortDimensions=1
  StPassCmprtMdCtrl_Md61_VCUCfg_Val : Outport  Port=308  OutDataTypeStr=boolean  PortDimensions=1
  StPassCmprtMdCtrl_Md62_VCUCfg_Val : Outport  Port=309  OutDataTypeStr=boolean  PortDimensions=1
  wires:
  AbgDplyBckp_Val/1 -> PreConitionRunnable_sys/1(AbgDplyBckp_Val_read)
  AbgDplyBckpV_Val/1 -> PreConitionRunnable_sys/2(AbgDplyBckpV_Val_read)
  AcsEntryPosLrnd_Val/1 -> PreConitionRunnable_sys/3(AcsEntryPosLrnd_Val_read)
  DrvStPosRclRspStat_Val/1 -> PreConitionRunnable_sys/4(DrvStPosRclRspStat_Val_read)
  EnergyMgLdShdRq_Val/1 -> PreConitionRunnable_sys/5(EnergyMgLdShdRq_Val_read)
  FamilyLtPosLrnd_Val/1 -> PreConitionRunnable_sys/6(FamilyLtPosLrnd_Val_read)
  FamilyRtPosLrnd_Val/1 -> PreConitionRunnable_sys/7(FamilyRtPosLrnd_Val_read)
  IfVeSMSeStNumConfig_Val/1 -> PreConitionRunnable_sys/8(IfVeSMSeStNumConfig_Val_read)
  IntimacyLPosLrnd_Val/1 -> PreConitionRunnable_sys/9(IntimacyLPosLrnd_Val_read)
  IntimacyRPosLrnd_Val/1 -> PreConitionRunnable_sys/10(IntimacyRPosLrnd_Val_read)
  Is2LStSwAct_Val/1 -> PreConitionRunnable_sys/11(Is2LStSwAct_Val_read)
  Is2RStSwAct_Val/1 -> PreConitionRunnable_sys/12(Is2RStSwAct_Val_read)
  Is3LStSwAct_Val/1 -> PreConitionRunnable_sys/13(Is3LStSwAct_Val_read)
  Is3RStSwAct_Val/1 -> PreConitionRunnable_sys/14(Is3RStSwAct_Val_read)
  IsDrvStSwAct_Val/1 -> PreConitionRunnable_sys/15(IsDrvStSwAct_Val_read)
  IsPasStSwAct_Val/1 -> PreConitionRunnable_sys/16(IsPasStSwAct_Val_read)
  LgrstCloseLtPosLrnd_Val/1 -> PreConitionRunnable_sys/17(LgrstCloseLtPosLrnd_Val_read)
  LgrstCloseRtPosLrnd_Val/1 -> PreConitionRunnable_sys/18(LgrstCloseRtPosLrnd_Val_read)
  LgrstOpenLtPosLrnd_Val/1 -> PreConitionRunnable_sys/19(LgrstOpenLtPosLrnd_Val_read)
  LgrstOpenRtPosLrnd_Val/1 -> PreConitionRunnable_sys/20(LgrstOpenRtPosLrnd_Val_read)
  LugLtPosLrnd_Val/1 -> PreConitionRunnable_sys/21(LugLtPosLrnd_Val_read)
  LugRtPosLrnd_Val/1 -> PreConitionRunnable_sys/22(LugRtPosLrnd_Val_read)
  LyingLtPosLrnd_Val/1 -> PreConitionRunnable_sys/23(LyingLtPosLrnd_Val_read)
  LyingRtPosLrnd_Val/1 -> PreConitionRunnable_sys/24(LyingRtPosLrnd_Val_read)
  MmryRclImpctDisRq_Val/1 -> PreConitionRunnable_sys/25(MmryRclImpctDisRq_Val_read)
  AcsExitPosLrnd_Val/1 -> PreConitionRunnable_sys/26(AcsExitPosLrnd_Val_read)
  PassStPosRclRspStat_Val/1 -> PreConitionRunnable_sys/27(PassStPosRclRspStat_Val_read)
  VIPLtPosLrnd_Val/1 -> PreConitionRunnable_sys/28(VIPLtPosLrnd_Val_read)
  SecRwLtStChldLkReq_Val/1 -> PreConitionRunnable_sys/29(SecRwLtStChldLkReq_Val_read)
  SecRwLtStPosRclRspStat_Val/1 -> PreConitionRunnable_sys/30(SecRwLtStPosRclRspStat_Val_read)
  VIPRtPosLrnd_Val/1 -> PreConitionRunnable_sys/31(VIPRtPosLrnd_Val_read)
  SecRwRtStChldLkReq_Val/1 -> PreConitionRunnable_sys/32(SecRwRtStChldLkReq_Val_read)
  SecRwRtStPosRclRspStat_Val/1 -> PreConitionRunnable_sys/33(SecRwRtStPosRclRspStat_Val_read)
  SysPwrMd_Val/1 -> PreConitionRunnable_sys/34(SysPwrMd_Val_read)
  SysPwrMdV_Val/1 -> PreConitionRunnable_sys/35(SysPwrMdV_Val_read)
  ThdRwCtStOccStatMSMSrc_Val/1 -> PreConitionRunnable_sys/36(ThdRwCtStOccStatMSMSrc_Val_read)
  RcvyLtPosLrnd_Val/1 -> PreConitionRunnable_sys/37(RcvyLtPosLrnd_Val_read)
  ThdRwLtStOccStatMSMSrc_Val/1 -> PreConitionRunnable_sys/38(ThdRwLtStOccStatMSMSrc_Val_read)
  ThdRwLtStPosRclRspStat_Val/1 -> PreConitionRunnable_sys/39(ThdRwLtStPosRclRspStat_Val_read)
  RcvyRtPosLrnd_Val/1 -> PreConitionRunnable_sys/40(RcvyRtPosLrnd_Val_read)
  ThdRwRtStOccStatMSMSrc_Val/1 -> PreConitionRunnable_sys/41(ThdRwRtStOccStatMSMSrc_Val_read)
  ThdRwRtStPosRclRspStat_Val/1 -> PreConitionRunnable_sys/42(ThdRwRtStPosRclRspStat_Val_read)
  VehMovState_Val/1 -> PreConitionRunnable_sys/43(VehMovState_Val_read)
  VehSpdAvgDrvn_Val/1 -> PreConitionRunnable_sys/44(VehSpdAvgDrvn_Val_read)
  VehSpdAvgDrvnV_Val/1 -> PreConitionRunnable_sys/45(VehSpdAvgDrvnV_Val_read)
  VeSignalLost2R_463_2L_Val/1 -> PreConitionRunnable_sys/46(VeSignalLost2R_463_2L_Val_read)
  VeSignalLost3L_468_2L_Val/1 -> PreConitionRunnable_sys/47(VeSignalLost3L_468_2L_Val_read)
  VeSignalLost3R_46C_2L_Val/1 -> PreConitionRunnable_sys/48(VeSignalLost3R_46C_2L_Val_read)
  VeSignalLostCODR_470_2L_Val/1 -> PreConitionRunnable_sys/49(VeSignalLostCODR_470_2L_Val_read)
  VeSignalLostDR_213_2L_Val/1 -> PreConitionRunnable_sys/50(VeSignalLostDR_213_2L_Val_read)
  VeSignalLostFireWall_1D2_2L_Val/1 -> PreConitionRunnable_sys/51(VeSignalLostFireWall_1D2_2L_Val_read)
  VeSignalLostSDM_195_2L_Val/1 -> PreConitionRunnable_sys/52(VeSignalLostSDM_195_2L_Val_read)
  VoltSts_Val/1 -> PreConitionRunnable_sys/53(VoltSts_Val_read)
  PreConitionRunnable_sys/1(AcsMdEntyAvl_Val_write) -> AcsMdEntyAvl_Val/1
  PreConitionRunnable_sys/2(AcsMdExtAvl_Val_write) -> AcsMdExtAvl_Val/1
  PreConitionRunnable_sys/3(CommCond_Val_write) -> CommCond_Val/1
  PreConitionRunnable_sys/4(CommExitCond_Val_write) -> CommExitCond_Val/1
  PreConitionRunnable_sys/5(CommExitCondwithSpeed_Val_write) -> CommExitCondwithSpeed_Val/1
  PreConitionRunnable_sys/6(DiagAbgDly_Val_write) -> DiagAbgDly_Val/1
  PreConitionRunnable_sys/7(DiagVehMovState_Val_write) -> DiagVehMovState_Val/1
  PreConitionRunnable_sys/8(DiagVehSpdAvgDrvn_Val_write) -> DiagVehSpdAvgDrvn_Val/1
  PreConitionRunnable_sys/9(FamilyMdLtAvl_Val_write) -> FamilyMdLtAvl_Val/1
  PreConitionRunnable_sys/10(FamilyMdRtAvl_Val_write) -> FamilyMdRtAvl_Val/1
  PreConitionRunnable_sys/11(HMIMd10Avl_2L_Val_write) -> HMIMd10Avl_2L_Val/1
  PreConitionRunnable_sys/12(HMIMd10Avl_2R_Val_write) -> HMIMd10Avl_2R_Val/1
  PreConitionRunnable_sys/13(HMIMd10Cfg_2L_Val_write) -> HMIMd10Cfg_2L_Val/1
  PreConitionRunnable_sys/14(HMIMd10Cfg_2R_Val_write) -> HMIMd10Cfg_2R_Val/1
  PreConitionRunnable_sys/15(HMIMd11Avl_2L_Val_write) -> HMIMd11Avl_2L_Val/1
  PreConitionRunnable_sys/16(HMIMd11Avl_2R_Val_write) -> HMIMd11Avl_2R_Val/1
  PreConitionRunnable_sys/17(HMIMd11Cfg_2L_Val_write) -> HMIMd11Cfg_2L_Val/1
  PreConitionRunnable_sys/18(HMIMd11Cfg_2R_Val_write) -> HMIMd11Cfg_2R_Val/1
  PreConitionRunnable_sys/19(HMIMd12Avl_2L_Val_write) -> HMIMd12Avl_2L_Val/1
  PreConitionRunnable_sys/20(HMIMd12Avl_2R_Val_write) -> HMIMd12Avl_2R_Val/1
  PreConitionRunnable_sys/21(HMIMd12Cfg_2L_Val_write) -> HMIMd12Cfg_2L_Val/1
  PreConitionRunnable_sys/22(HMIMd12Cfg_2R_Val_write) -> HMIMd12Cfg_2R_Val/1
  PreConitionRunnable_sys/23(HMIMd13Avl_2L_Val_write) -> HMIMd13Avl_2L_Val/1
  PreConitionRunnable_sys/24(HMIMd13Avl_2R_Val_write) -> HMIMd13Avl_2R_Val/1
  PreConitionRunnable_sys/25(HMIMd13Cfg_2L_Val_write) -> HMIMd13Cfg_2L_Val/1
  PreConitionRunnable_sys/26(HMIMd13Cfg_2R_Val_write) -> HMIMd13Cfg_2R_Val/1
  PreConitionRunnable_sys/27(HMIMd14Avl_2L_Val_write) -> HMIMd14Avl_2L_Val/1
  PreConitionRunnable_sys/28(HMIMd14Avl_2R_Val_write) -> HMIMd14Avl_2R_Val/1
  PreConitionRunnable_sys/29(HMIMd14Cfg_2L_Val_write) -> HMIMd14Cfg_2L_Val/1
  PreConitionRunnable_sys/30(HMIMd14Cfg_2R_Val_write) -> HMIMd14Cfg_2R_Val/1
  PreConitionRunnable_sys/31(HMIMd15Avl_2L_Val_write) -> HMIMd15Avl_2L_Val/1
  PreConitionRunnable_sys/32(HMIMd15Avl_2R_Val_write) -> HMIMd15Avl_2R_Val/1
  PreConitionRunnable_sys/33(HMIMd15Cfg_2L_Val_write) -> HMIMd15Cfg_2L_Val/1
  PreConitionRunnable_sys/34(HMIMd15Cfg_2R_Val_write) -> HMIMd15Cfg_2R_Val/1
  PreConitionRunnable_sys/35(HMIMd16Avl_2L_Val_write) -> HMIMd16Avl_2L_Val/1
  PreConitionRunnable_sys/36(HMIMd16Avl_2R_Val_write) -> HMIMd16Avl_2R_Val/1
  PreConitionRunnable_sys/37(HMIMd16Cfg_2L_Val_write) -> HMIMd16Cfg_2L_Val/1
  PreConitionRunnable_sys/38(HMIMd16Cfg_2R_Val_write) -> HMIMd16Cfg_2R_Val/1
  PreConitionRunnable_sys/39(HMIMd17Avl_2L_Val_write) -> HMIMd17Avl_2L_Val/1
  PreConitionRunnable_sys/40(HMIMd17Avl_2R_Val_write) -> HMIMd17Avl_2R_Val/1
  PreConitionRunnable_sys/41(HMIMd17Cfg_2L_Val_write) -> HMIMd17Cfg_2L_Val/1
  PreConitionRunnable_sys/42(HMIMd17Cfg_2R_Val_write) -> HMIMd17Cfg_2R_Val/1
  PreConitionRunnable_sys/43(HMIMd18Avl_2L_Val_write) -> HMIMd18Avl_2L_Val/1
  PreConitionRunnable_sys/44(HMIMd18Avl_2R_Val_write) -> HMIMd18Avl_2R_Val/1
  PreConitionRunnable_sys/45(HMIMd18Cfg_2L_Val_write) -> HMIMd18Cfg_2L_Val/1
  PreConitionRunnable_sys/46(HMIMd18Cfg_2R_Val_write) -> HMIMd18Cfg_2R_Val/1
  PreConitionRunnable_sys/47(HMIMd19Avl_2L_Val_write) -> HMIMd19Avl_2L_Val/1
  PreConitionRunnable_sys/48(HMIMd19Avl_2R_Val_write) -> HMIMd19Avl_2R_Val/1
  PreConitionRunnable_sys/49(HMIMd19Cfg_2L_Val_write) -> HMIMd19Cfg_2L_Val/1
  PreConitionRunnable_sys/50(HMIMd19Cfg_2R_Val_write) -> HMIMd19Cfg_2R_Val/1
  PreConitionRunnable_sys/51(HMIMd1Avl_2L_Val_write) -> HMIMd1Avl_2L_Val/1
  PreConitionRunnable_sys/52(HMIMd1Avl_2R_Val_write) -> HMIMd1Avl_2R_Val/1
  PreConitionRunnable_sys/53(HMIMd1Cfg_2L_Val_write) -> HMIMd1Cfg_2L_Val/1
  PreConitionRunnable_sys/54(HMIMd1Cfg_2R_Val_write) -> HMIMd1Cfg_2R_Val/1
  PreConitionRunnable_sys/55(HMIMd20Avl_2L_Val_write) -> HMIMd20Avl_2L_Val/1
  PreConitionRunnable_sys/56(HMIMd20Avl_2R_Val_write) -> HMIMd20Avl_2R_Val/1
  PreConitionRunnable_sys/57(HMIMd20Cfg_2L_Val_write) -> HMIMd20Cfg_2L_Val/1
  PreConitionRunnable_sys/58(HMIMd20Cfg_2R_Val_write) -> HMIMd20Cfg_2R_Val/1
  PreConitionRunnable_sys/59(HMIMd21Avl_2L_Val_write) -> HMIMd21Avl_2L_Val/1
  PreConitionRunnable_sys/60(HMIMd21Avl_2R_Val_write) -> HMIMd21Avl_2R_Val/1
  PreConitionRunnable_sys/61(HMIMd21Cfg_2L_Val_write) -> HMIMd21Cfg_2L_Val/1
  PreConitionRunnable_sys/62(HMIMd21Cfg_2R_Val_write) -> HMIMd21Cfg_2R_Val/1
  PreConitionRunnable_sys/63(HMIMd22Avl_2L_Val_write) -> HMIMd22Avl_2L_Val/1
  PreConitionRunnable_sys/64(HMIMd22Avl_2R_Val_write) -> HMIMd22Avl_2R_Val/1
  PreConitionRunnable_sys/65(HMIMd22Cfg_2L_Val_write) -> HMIMd22Cfg_2L_Val/1
  PreConitionRunnable_sys/66(HMIMd22Cfg_2R_Val_write) -> HMIMd22Cfg_2R_Val/1
  PreConitionRunnable_sys/67(HMIMd23Avl_2L_Val_write) -> HMIMd23Avl_2L_Val/1
  PreConitionRunnable_sys/68(HMIMd23Avl_2R_Val_write) -> HMIMd23Avl_2R_Val/1
  PreConitionRunnable_sys/69(HMIMd23Cfg_2L_Val_write) -> HMIMd23Cfg_2L_Val/1
  PreConitionRunnable_sys/70(HMIMd23Cfg_2R_Val_write) -> HMIMd23Cfg_2R_Val/1
  PreConitionRunnable_sys/71(HMIMd24Avl_2L_Val_write) -> HMIMd24Avl_2L_Val/1
  PreConitionRunnable_sys/72(HMIMd24Avl_2R_Val_write) -> HMIMd24Avl_2R_Val/1
  PreConitionRunnable_sys/73(HMIMd24Cfg_2L_Val_write) -> HMIMd24Cfg_2L_Val/1
  PreConitionRunnable_sys/74(HMIMd24Cfg_2R_Val_write) -> HMIMd24Cfg_2R_Val/1
  PreConitionRunnable_sys/75(HMIMd25Avl_2L_Val_write) -> HMIMd25Avl_2L_Val/1
  PreConitionRunnable_sys/76(HMIMd25Avl_2R_Val_write) -> HMIMd25Avl_2R_Val/1
  PreConitionRunnable_sys/77(HMIMd25Cfg_2L_Val_write) -> HMIMd25Cfg_2L_Val/1
  PreConitionRunnable_sys/78(HMIMd25Cfg_2R_Val_write) -> HMIMd25Cfg_2R_Val/1
  PreConitionRunnable_sys/79(HMIMd26Avl_2L_Val_write) -> HMIMd26Avl_2L_Val/1
  PreConitionRunnable_sys/80(HMIMd26Avl_2R_Val_write) -> HMIMd26Avl_2R_Val/1
  PreConitionRunnable_sys/81(HMIMd26Cfg_2L_Val_write) -> HMIMd26Cfg_2L_Val/1
  PreConitionRunnable_sys/82(HMIMd26Cfg_2R_Val_write) -> HMIMd26Cfg_2R_Val/1
  PreConitionRunnable_sys/83(HMIMd27Avl_2L_Val_write) -> HMIMd27Avl_2L_Val/1
  PreConitionRunnable_sys/84(HMIMd27Avl_2R_Val_write) -> HMIMd27Avl_2R_Val/1
  PreConitionRunnable_sys/85(HMIMd27Cfg_2L_Val_write) -> HMIMd27Cfg_2L_Val/1
  PreConitionRunnable_sys/86(HMIMd27Cfg_2R_Val_write) -> HMIMd27Cfg_2R_Val/1
  PreConitionRunnable_sys/87(HMIMd28Avl_2L_Val_write) -> HMIMd28Avl_2L_Val/1
  PreConitionRunnable_sys/88(HMIMd28Avl_2R_Val_write) -> HMIMd28Avl_2R_Val/1
  PreConitionRunnable_sys/89(HMIMd28Cfg_2L_Val_write) -> HMIMd28Cfg_2L_Val/1
  PreConitionRunnable_sys/90(HMIMd28Cfg_2R_Val_write) -> HMIMd28Cfg_2R_Val/1
  PreConitionRunnable_sys/91(HMIMd29Avl_2L_Val_write) -> HMIMd29Avl_2L_Val/1
  PreConitionRunnable_sys/92(HMIMd29Avl_2R_Val_write) -> HMIMd29Avl_2R_Val/1
  PreConitionRunnable_sys/93(HMIMd29Cfg_2L_Val_write) -> HMIMd29Cfg_2L_Val/1
  PreConitionRunnable_sys/94(HMIMd29Cfg_2R_Val_write) -> HMIMd29Cfg_2R_Val/1
  PreConitionRunnable_sys/95(HMIMd2Avl_2L_Val_write) -> HMIMd2Avl_2L_Val/1
  PreConitionRunnable_sys/96(HMIMd2Avl_2R_Val_write) -> HMIMd2Avl_2R_Val/1
  PreConitionRunnable_sys/97(HMIMd2Cfg_2L_Val_write) -> HMIMd2Cfg_2L_Val/1
  PreConitionRunnable_sys/98(HMIMd2Cfg_2R_Val_write) -> HMIMd2Cfg_2R_Val/1
  PreConitionRunnable_sys/99(HMIMd30Avl_2L_Val_write) -> HMIMd30Avl_2L_Val/1
  PreConitionRunnable_sys/100(HMIMd30Avl_2R_Val_write) -> HMIMd30Avl_2R_Val/1
  PreConitionRunnable_sys/101(HMIMd30Cfg_2L_Val_write) -> HMIMd30Cfg_2L_Val/1
  PreConitionRunnable_sys/102(HMIMd30Cfg_2R_Val_write) -> HMIMd30Cfg_2R_Val/1
  PreConitionRunnable_sys/103(HMIMd31Avl_2L_Val_write) -> HMIMd31Avl_2L_Val/1
  PreConitionRunnable_sys/104(HMIMd31Avl_2R_Val_write) -> HMIMd31Avl_2R_Val/1
  PreConitionRunnable_sys/105(HMIMd31Cfg_2L_Val_write) -> HMIMd31Cfg_2L_Val/1
  PreConitionRunnable_sys/106(HMIMd31Cfg_2R_Val_write) -> HMIMd31Cfg_2R_Val/1
  PreConitionRunnable_sys/107(HMIMd32Avl_2L_Val_write) -> HMIMd32Avl_2L_Val/1
  PreConitionRunnable_sys/108(HMIMd32Avl_2R_Val_write) -> HMIMd32Avl_2R_Val/1
  PreConitionRunnable_sys/109(HMIMd32Cfg_2L_Val_write) -> HMIMd32Cfg_2L_Val/1
  PreConitionRunnable_sys/110(HMIMd32Cfg_2R_Val_write) -> HMIMd32Cfg_2R_Val/1
  PreConitionRunnable_sys/111(HMIMd3Avl_2L_Val_write) -> HMIMd3Avl_2L_Val/1
  PreConitionRunnable_sys/112(HMIMd3Avl_2R_Val_write) -> HMIMd3Avl_2R_Val/1
  PreConitionRunnable_sys/113(HMIMd3Cfg_2L_Val_write) -> HMIMd3Cfg_2L_Val/1
  PreConitionRunnable_sys/114(HMIMd3Cfg_2R_Val_write) -> HMIMd3Cfg_2R_Val/1
  PreConitionRunnable_sys/115(HMIMd4Avl_2L_Val_write) -> HMIMd4Avl_2L_Val/1
  PreConitionRunnable_sys/116(HMIMd4Avl_2R_Val_write) -> HMIMd4Avl_2R_Val/1
  PreConitionRunnable_sys/117(HMIMd4Cfg_2L_Val_write) -> HMIMd4Cfg_2L_Val/1
  PreConitionRunnable_sys/118(HMIMd4Cfg_2R_Val_write) -> HMIMd4Cfg_2R_Val/1
  PreConitionRunnable_sys/119(HMIMd5Avl_2L_Val_write) -> HMIMd5Avl_2L_Val/1
  PreConitionRunnable_sys/120(HMIMd5Avl_2R_Val_write) -> HMIMd5Avl_2R_Val/1
  PreConitionRunnable_sys/121(HMIMd5Cfg_2L_Val_write) -> HMIMd5Cfg_2L_Val/1
  PreConitionRunnable_sys/122(HMIMd5Cfg_2R_Val_write) -> HMIMd5Cfg_2R_Val/1
  PreConitionRunnable_sys/123(HMIMd6Avl_2L_Val_write) -> HMIMd6Avl_2L_Val/1
  PreConitionRunnable_sys/124(HMIMd6Avl_2R_Val_write) -> HMIMd6Avl_2R_Val/1
  PreConitionRunnable_sys/125(HMIMd6Cfg_2L_Val_write) -> HMIMd6Cfg_2L_Val/1
  PreConitionRunnable_sys/126(HMIMd6Cfg_2R_Val_write) -> HMIMd6Cfg_2R_Val/1
  PreConitionRunnable_sys/127(HMIMd7Avl_2L_Val_write) -> HMIMd7Avl_2L_Val/1
  PreConitionRunnable_sys/128(HMIMd7Avl_2R_Val_write) -> HMIMd7Avl_2R_Val/1
  PreConitionRunnable_sys/129(HMIMd7Cfg_2L_Val_write) -> HMIMd7Cfg_2L_Val/1
  PreConitionRunnable_sys/130(HMIMd7Cfg_2R_Val_write) -> HMIMd7Cfg_2R_Val/1
  PreConitionRunnable_sys/131(HMIMd8Avl_2L_Val_write) -> HMIMd8Avl_2L_Val/1
  PreConitionRunnable_sys/132(HMIMd8Avl_2R_Val_write) -> HMIMd8Avl_2R_Val/1
  PreConitionRunnable_sys/133(HMIMd8Cfg_2L_Val_write) -> HMIMd8Cfg_2L_Val/1
  PreConitionRunnable_sys/134(HMIMd8Cfg_2R_Val_write) -> HMIMd8Cfg_2R_Val/1
  PreConitionRunnable_sys/135(HMIMd9Avl_2L_Val_write) -> HMIMd9Avl_2L_Val/1
  PreConitionRunnable_sys/136(HMIMd9Avl_2R_Val_write) -> HMIMd9Avl_2R_Val/1
  PreConitionRunnable_sys/137(HMIMd9Cfg_2L_Val_write) -> HMIMd9Cfg_2L_Val/1
  PreConitionRunnable_sys/138(HMIMd9Cfg_2R_Val_write) -> HMIMd9Cfg_2R_Val/1
  PreConitionRunnable_sys/139(IntimacyLMdAvl_Val_write) -> IntimacyLMdAvl_Val/1
  PreConitionRunnable_sys/140(IntimacyRMdAvl_Val_write) -> IntimacyRMdAvl_Val/1
  PreConitionRunnable_sys/141(LgrstCloseLtMdAvl_Val_write) -> LgrstCloseLtMdAvl_Val/1
  PreConitionRunnable_sys/142(LgrstCloseRtMdAvl_Val_write) -> LgrstCloseRtMdAvl_Val/1
  PreConitionRunnable_sys/143(LgrstOpenLtMdAvl_Val_write) -> LgrstOpenLtMdAvl_Val/1
  PreConitionRunnable_sys/144(LgrstOpenRtMdAvl_Val_write) -> LgrstOpenRtMdAvl_Val/1
  PreConitionRunnable_sys/145(LugMdLtAvl_Val_write) -> LugMdLtAvl_Val/1
  PreConitionRunnable_sys/146(LugMdRtAvl_Val_write) -> LugMdRtAvl_Val/1
  PreConitionRunnable_sys/147(LyingMdLtAvl_Val_write) -> LyingMdLtAvl_Val/1
  PreConitionRunnable_sys/148(LyingMdRtAvl_Val_write) -> LyingMdRtAvl_Val/1
  PreConitionRunnable_sys/149(PwrMdChked_Val_write) -> PwrMdChked_Val/1
  PreConitionRunnable_sys/150(RcvyMdLtAvl_Val_write) -> RcvyMdLtAvl_Val/1
  PreConitionRunnable_sys/151(RcvyMdRtAvl_Val_write) -> RcvyMdRtAvl_Val/1
  PreConitionRunnable_sys/152(StPassCmprtMdCtrl_Md1_VCUAvl_Val_write) -> StPassCmprtMdCtrl_Md1_VCUAvl_Val/1
  PreConitionRunnable_sys/153(StPassCmprtMdCtrl_Md1_VCUCfg_Val_write) -> StPassCmprtMdCtrl_Md1_VCUCfg_Val/1
  PreConitionRunnable_sys/154(StPassCmprtMdCtrl_Md10_VCUAvl_Val_write) -> StPassCmprtMdCtrl_Md10_VCUAvl_Val/1
  PreConitionRunnable_sys/155(StPassCmprtMdCtrl_Md10_VCUCfg_Val_write) -> StPassCmprtMdCtrl_Md10_VCUCfg_Val/1
  PreConitionRunnable_sys/156(StPassCmprtMdCtrl_Md11_VCUAvl_Val_write) -> StPassCmprtMdCtrl_Md11_VCUAvl_Val/1
  PreConitionRunnable_sys/157(StPassCmprtMdCtrl_Md11_VCUCfg_Val_write) -> StPassCmprtMdCtrl_Md11_VCUCfg_Val/1
  PreConitionRunnable_sys/158(StPassCmprtMdCtrl_Md12_VCUAvl_Val_write) -> StPassCmprtMdCtrl_Md12_VCUAvl_Val/1
  PreConitionRunnable_sys/159(StPassCmprtMdCtrl_Md12_VCUCfg_Val_write) -> StPassCmprtMdCtrl_Md12_VCUCfg_Val/1
  PreConitionRunnable_sys/160(StPassCmprtMdCtrl_Md13_VCUAvl_Val_write) -> StPassCmprtMdCtrl_Md13_VCUAvl_Val/1
  PreConitionRunnable_sys/161(StPassCmprtMdCtrl_Md13_VCUCfg_Val_write) -> StPassCmprtMdCtrl_Md13_VCUCfg_Val/1
  PreConitionRunnable_sys/162(StPassCmprtMdCtrl_Md14_VCUAvl_Val_write) -> StPassCmprtMdCtrl_Md14_VCUAvl_Val/1
  PreConitionRunnable_sys/163(StPassCmprtMdCtrl_Md14_VCUCfg_Val_write) -> StPassCmprtMdCtrl_Md14_VCUCfg_Val/1
  PreConitionRunnable_sys/164(StPassCmprtMdCtrl_Md15_VCUAvl_Val_write) -> StPassCmprtMdCtrl_Md15_VCUAvl_Val/1
  PreConitionRunnable_sys/165(StPassCmprtMdCtrl_Md15_VCUCfg_Val_write) -> StPassCmprtMdCtrl_Md15_VCUCfg_Val/1
  PreConitionRunnable_sys/166(StPassCmprtMdCtrl_Md16_VCUAvl_Val_write) -> StPassCmprtMdCtrl_Md16_VCUAvl_Val/1
  PreConitionRunnable_sys/167(StPassCmprtMdCtrl_Md16_VCUCfg_Val_write) -> StPassCmprtMdCtrl_Md16_VCUCfg_Val/1
  PreConitionRunnable_sys/168(StPassCmprtMdCtrl_Md17_VCUAvl_Val_write) -> StPassCmprtMdCtrl_Md17_VCUAvl_Val/1
  PreConitionRunnable_sys/169(StPassCmprtMdCtrl_Md17_VCUCfg_Val_write) -> StPassCmprtMdCtrl_Md17_VCUCfg_Val/1
  PreConitionRunnable_sys/170(StPassCmprtMdCtrl_Md18_VCUAvl_Val_write) -> StPassCmprtMdCtrl_Md18_VCUAvl_Val/1
  PreConitionRunnable_sys/171(StPassCmprtMdCtrl_Md18_VCUCfg_Val_write) -> StPassCmprtMdCtrl_Md18_VCUCfg_Val/1
  PreConitionRunnable_sys/172(StPassCmprtMdCtrl_Md19_VCUAvl_Val_write) -> StPassCmprtMdCtrl_Md19_VCUAvl_Val/1
  PreConitionRunnable_sys/173(StPassCmprtMdCtrl_Md19_VCUCfg_Val_write) -> StPassCmprtMdCtrl_Md19_VCUCfg_Val/1
  PreConitionRunnable_sys/174(StPassCmprtMdCtrl_Md2_VCUAvl_Val_write) -> StPassCmprtMdCtrl_Md2_VCUAvl_Val/1
  PreConitionRunnable_sys/175(StPassCmprtMdCtrl_Md2_VCUCfg_Val_write) -> StPassCmprtMdCtrl_Md2_VCUCfg_Val/1
  PreConitionRunnable_sys/176(StPassCmprtMdCtrl_Md20_VCUAvl_Val_write) -> StPassCmprtMdCtrl_Md20_VCUAvl_Val/1
  PreConitionRunnable_sys/177(StPassCmprtMdCtrl_Md20_VCUCfg_Val_write) -> StPassCmprtMdCtrl_Md20_VCUCfg_Val/1
  PreConitionRunnable_sys/178(StPassCmprtMdCtrl_Md21_VCUAvl_Val_write) -> StPassCmprtMdCtrl_Md21_VCUAvl_Val/1
  PreConitionRunnable_sys/179(StPassCmprtMdCtrl_Md21_VCUCfg_Val_write) -> StPassCmprtMdCtrl_Md21_VCUCfg_Val/1
  PreConitionRunnable_sys/180(StPassCmprtMdCtrl_Md22_VCUAvl_Val_write) -> StPassCmprtMdCtrl_Md22_VCUAvl_Val/1
  PreConitionRunnable_sys/181(StPassCmprtMdCtrl_Md22_VCUCfg_Val_write) -> StPassCmprtMdCtrl_Md22_VCUCfg_Val/1
  PreConitionRunnable_sys/182(StPassCmprtMdCtrl_Md23_VCUAvl_Val_write) -> StPassCmprtMdCtrl_Md23_VCUAvl_Val/1
  PreConitionRunnable_sys/183(StPassCmprtMdCtrl_Md23_VCUCfg_Val_write) -> StPassCmprtMdCtrl_Md23_VCUCfg_Val/1
  PreConitionRunnable_sys/184(StPassCmprtMdCtrl_Md24_VCUAvl_Val_write) -> StPassCmprtMdCtrl_Md24_VCUAvl_Val/1
  PreConitionRunnable_sys/185(StPassCmprtMdCtrl_Md24_VCUCfg_Val_write) -> StPassCmprtMdCtrl_Md24_VCUCfg_Val/1
  PreConitionRunnable_sys/186(StPassCmprtMdCtrl_Md25_VCUAvl_Val_write) -> StPassCmprtMdCtrl_Md25_VCUAvl_Val/1
  PreConitionRunnable_sys/187(StPassCmprtMdCtrl_Md25_VCUCfg_Val_write) -> StPassCmprtMdCtrl_Md25_VCUCfg_Val/1
  PreConitionRunnable_sys/188(StPassCmprtMdCtrl_Md26_VCUAvl_Val_write) -> StPassCmprtMdCtrl_Md26_VCUAvl_Val/1
  PreConitionRunnable_sys/189(StPassCmprtMdCtrl_Md26_VCUCfg_Val_write) -> StPassCmprtMdCtrl_Md26_VCUCfg_Val/1
  PreConitionRunnable_sys/190(StPassCmprtMdCtrl_Md27_VCUAvl_Val_write) -> StPassCmprtMdCtrl_Md27_VCUAvl_Val/1
  PreConitionRunnable_sys/191(StPassCmprtMdCtrl_Md27_VCUCfg_Val_write) -> StPassCmprtMdCtrl_Md27_VCUCfg_Val/1
  PreConitionRunnable_sys/192(StPassCmprtMdCtrl_Md28_VCUAvl_Val_write) -> StPassCmprtMdCtrl_Md28_VCUAvl_Val/1
  PreConitionRunnable_sys/193(StPassCmprtMdCtrl_Md28_VCUCfg_Val_write) -> StPassCmprtMdCtrl_Md28_VCUCfg_Val/1
  PreConitionRunnable_sys/194(StPassCmprtMdCtrl_Md29_VCUAvl_Val_write) -> StPassCmprtMdCtrl_Md29_VCUAvl_Val/1
  PreConitionRunnable_sys/195(StPassCmprtMdCtrl_Md29_VCUCfg_Val_write) -> StPassCmprtMdCtrl_Md29_VCUCfg_Val/1
  PreConitionRunnable_sys/196(StPassCmprtMdCtrl_Md3_VCUAvl_Val_write) -> StPassCmprtMdCtrl_Md3_VCUAvl_Val/1
  PreConitionRunnable_sys/197(StPassCmprtMdCtrl_Md3_VCUCfg_Val_write) -> StPassCmprtMdCtrl_Md3_VCUCfg_Val/1
  PreConitionRunnable_sys/198(StPassCmprtMdCtrl_Md30_VCUAvl_Val_write) -> StPassCmprtMdCtrl_Md30_VCUAvl_Val/1
  PreConitionRunnable_sys/199(StPassCmprtMdCtrl_Md30_VCUCfg_Val_write) -> StPassCmprtMdCtrl_Md30_VCUCfg_Val/1
  PreConitionRunnable_sys/200(StPassCmprtMdCtrl_Md31_VCUAvl_Val_write) -> StPassCmprtMdCtrl_Md31_VCUAvl_Val/1
  PreConitionRunnable_sys/201(StPassCmprtMdCtrl_Md31_VCUCfg_Val_write) -> StPassCmprtMdCtrl_Md31_VCUCfg_Val/1
  PreConitionRunnable_sys/202(StPassCmprtMdCtrl_Md32_VCUAvl_Val_write) -> StPassCmprtMdCtrl_Md32_VCUAvl_Val/1
  PreConitionRunnable_sys/203(StPassCmprtMdCtrl_Md32_VCUCfg_Val_write) -> StPassCmprtMdCtrl_Md32_VCUCfg_Val/1
  PreConitionRunnable_sys/204(StPassCmprtMdCtrl_Md4_VCUAvl_Val_write) -> StPassCmprtMdCtrl_Md4_VCUAvl_Val/1
  PreConitionRunnable_sys/205(StPassCmprtMdCtrl_Md4_VCUCfg_Val_write) -> StPassCmprtMdCtrl_Md4_VCUCfg_Val/1
  PreConitionRunnable_sys/206(StPassCmprtMdCtrl_Md5_VCUAvl_Val_write) -> StPassCmprtMdCtrl_Md5_VCUAvl_Val/1
  PreConitionRunnable_sys/207(StPassCmprtMdCtrl_Md5_VCUCfg_Val_write) -> StPassCmprtMdCtrl_Md5_VCUCfg_Val/1
  PreConitionRunnable_sys/208(StPassCmprtMdCtrl_Md6_VCUAvl_Val_write) -> StPassCmprtMdCtrl_Md6_VCUAvl_Val/1
  PreConitionRunnable_sys/209(StPassCmprtMdCtrl_Md6_VCUCfg_Val_write) -> StPassCmprtMdCtrl_Md6_VCUCfg_Val/1
  PreConitionRunnable_sys/210(StPassCmprtMdCtrl_Md7_VCUAvl_Val_write) -> StPassCmprtMdCtrl_Md7_VCUAvl_Val/1
  PreConitionRunnable_sys/211(StPassCmprtMdCtrl_Md7_VCUCfg_Val_write) -> StPassCmprtMdCtrl_Md7_VCUCfg_Val/1
  PreConitionRunnable_sys/212(StPassCmprtMdCtrl_Md8_VCUAvl_Val_write) -> StPassCmprtMdCtrl_Md8_VCUAvl_Val/1
  PreConitionRunnable_sys/213(StPassCmprtMdCtrl_Md8_VCUCfg_Val_write) -> StPassCmprtMdCtrl_Md8_VCUCfg_Val/1
  PreConitionRunnable_sys/214(StPassCmprtMdCtrl_Md9_VCUAvl_Val_write) -> StPassCmprtMdCtrl_Md9_VCUAvl_Val/1
  PreConitionRunnable_sys/215(StPassCmprtMdCtrl_Md9_VCUCfg_Val_write) -> StPassCmprtMdCtrl_Md9_VCUCfg_Val/1
  PreConitionRunnable_sys/216(StPassCmprtMdRfCtrlSwCstStAvl_Val_write) -> StPassCmprtMdRfCtrlSwCstStAvl_Val/1
  PreConitionRunnable_sys/217(StSrvAvl_Md1_Val_write) -> StSrvAvl_Md1_Val/1
  PreConitionRunnable_sys/218(StSrvAvl_Md10_Val_write) -> StSrvAvl_Md10_Val/1
  PreConitionRunnable_sys/219(StSrvAvl_Md11_Val_write) -> StSrvAvl_Md11_Val/1
  PreConitionRunnable_sys/221(StSrvAvl_Md12_Val_write) -> StSrvAvl_Md12_Val/1
  PreConitionRunnable_sys/220(StSrvAvl_Md13_Val_write) -> StSrvAvl_Md13_Val/1
  PreConitionRunnable_sys/222(StSrvAvl_Md14_Val_write) -> StSrvAvl_Md14_Val/1
  PreConitionRunnable_sys/223(StSrvAvl_Md15_Val_write) -> StSrvAvl_Md15_Val/1
  PreConitionRunnable_sys/224(StSrvAvl_Md16_Val_write) -> StSrvAvl_Md16_Val/1
  PreConitionRunnable_sys/225(StSrvAvl_Md17_Val_write) -> StSrvAvl_Md17_Val/1
  PreConitionRunnable_sys/226(StSrvAvl_Md18_Val_write) -> StSrvAvl_Md18_Val/1
  PreConitionRunnable_sys/227(StSrvAvl_Md19_Val_write) -> StSrvAvl_Md19_Val/1
  PreConitionRunnable_sys/228(StSrvAvl_Md2_Val_write) -> StSrvAvl_Md2_Val/1
  PreConitionRunnable_sys/229(StSrvAvl_Md20_Val_write) -> StSrvAvl_Md20_Val/1
  PreConitionRunnable_sys/230(StSrvAvl_Md21_Val_write) -> StSrvAvl_Md21_Val/1
  PreConitionRunnable_sys/231(StSrvAvl_Md22_Val_write) -> StSrvAvl_Md22_Val/1
  PreConitionRunnable_sys/232(StSrvAvl_Md23_Val_write) -> StSrvAvl_Md23_Val/1
  PreConitionRunnable_sys/233(StSrvAvl_Md24_Val_write) -> StSrvAvl_Md24_Val/1
  PreConitionRunnable_sys/234(StSrvAvl_Md25_Val_write) -> StSrvAvl_Md25_Val/1
  PreConitionRunnable_sys/235(StSrvAvl_Md26_Val_write) -> StSrvAvl_Md26_Val/1
  PreConitionRunnable_sys/236(StSrvAvl_Md27_Val_write) -> StSrvAvl_Md27_Val/1
  PreConitionRunnable_sys/237(StSrvAvl_Md28_Val_write) -> StSrvAvl_Md28_Val/1
  PreConitionRunnable_sys/238(StSrvAvl_Md29_Val_write) -> StSrvAvl_Md29_Val/1
  PreConitionRunnable_sys/239(StSrvAvl_Md3_Val_write) -> StSrvAvl_Md3_Val/1
  PreConitionRunnable_sys/240(StSrvAvl_Md30_Val_write) -> StSrvAvl_Md30_Val/1
  PreConitionRunnable_sys/241(StSrvAvl_Md31_Val_write) -> StSrvAvl_Md31_Val/1
  PreConitionRunnable_sys/242(StSrvAvl_Md32_Val_write) -> StSrvAvl_Md32_Val/1
  PreConitionRunnable_sys/243(StSrvAvl_Md4_Val_write) -> StSrvAvl_Md4_Val/1
  PreConitionRunnable_sys/244(StSrvAvl_Md5_Val_write) -> StSrvAvl_Md5_Val/1
  PreConitionRunnable_sys/245(StSrvAvl_Md6_Val_write) -> StSrvAvl_Md6_Val/1
  PreConitionRunnable_sys/246(StSrvAvl_Md7_Val_write) -> StSrvAvl_Md7_Val/1
  PreConitionRunnable_sys/247(StSrvAvl_Md8_Val_write) -> StSrvAvl_Md8_Val/1
  PreConitionRunnable_sys/248(StSrvAvl_Md9_Val_write) -> StSrvAvl_Md9_Val/1
  PreConitionRunnable_sys/249(StSrvCfg_Md1_Val_write) -> StSrvCfg_Md1_Val/1
  PreConitionRunnable_sys/250(StSrvCfg_Md10_Val_write) -> StSrvCfg_Md10_Val/1
  PreConitionRunnable_sys/251(StSrvCfg_Md11_Val_write) -> StSrvCfg_Md11_Val/1
  PreConitionRunnable_sys/252(StSrvCfg_Md12_Val_write) -> StSrvCfg_Md12_Val/1
  PreConitionRunnable_sys/253(StSrvCfg_Md13_Val_write) -> StSrvCfg_Md13_Val/1
  PreConitionRunnable_sys/254(StSrvCfg_Md14_Val_write) -> StSrvCfg_Md14_Val/1
  PreConitionRunnable_sys/255(StSrvCfg_Md15_Val_write) -> StSrvCfg_Md15_Val/1
  PreConitionRunnable_sys/256(StSrvCfg_Md16_Val_write) -> StSrvCfg_Md16_Val/1
  PreConitionRunnable_sys/257(StSrvCfg_Md17_Val_write) -> StSrvCfg_Md17_Val/1
  PreConitionRunnable_sys/258(StSrvCfg_Md18_Val_write) -> StSrvCfg_Md18_Val/1
  PreConitionRunnable_sys/259(StSrvCfg_Md19_Val_write) -> StSrvCfg_Md19_Val/1
  PreConitionRunnable_sys/260(StSrvCfg_Md2_Val_write) -> StSrvCfg_Md2_Val/1
  PreConitionRunnable_sys/261(StSrvCfg_Md20_Val_write) -> StSrvCfg_Md20_Val/1
  PreConitionRunnable_sys/262(StSrvCfg_Md21_Val_write) -> StSrvCfg_Md21_Val/1
  PreConitionRunnable_sys/263(StSrvCfg_Md22_Val_write) -> StSrvCfg_Md22_Val/1
  PreConitionRunnable_sys/264(StSrvCfg_Md23_Val_write) -> StSrvCfg_Md23_Val/1
  PreConitionRunnable_sys/265(StSrvCfg_Md24_Val_write) -> StSrvCfg_Md24_Val/1
  PreConitionRunnable_sys/266(StSrvCfg_Md25_Val_write) -> StSrvCfg_Md25_Val/1
  PreConitionRunnable_sys/267(StSrvCfg_Md26_Val_write) -> StSrvCfg_Md26_Val/1
  PreConitionRunnable_sys/268(StSrvCfg_Md27_Val_write) -> StSrvCfg_Md27_Val/1
  PreConitionRunnable_sys/269(StSrvCfg_Md28_Val_write) -> StSrvCfg_Md28_Val/1
  PreConitionRunnable_sys/270(StSrvCfg_Md29_Val_write) -> StSrvCfg_Md29_Val/1
  PreConitionRunnable_sys/271(StSrvCfg_Md3_Val_write) -> StSrvCfg_Md3_Val/1
  PreConitionRunnable_sys/272(StSrvCfg_Md30_Val_write) -> StSrvCfg_Md30_Val/1
  PreConitionRunnable_sys/273(StSrvCfg_Md31_Val_write) -> StSrvCfg_Md31_Val/1
  PreConitionRunnable_sys/274(StSrvCfg_Md32_Val_write) -> StSrvCfg_Md32_Val/1
  PreConitionRunnable_sys/275(StSrvCfg_Md4_Val_write) -> StSrvCfg_Md4_Val/1
  PreConitionRunnable_sys/276(StSrvCfg_Md5_Val_write) -> StSrvCfg_Md5_Val/1
  PreConitionRunnable_sys/277(StSrvCfg_Md6_Val_write) -> StSrvCfg_Md6_Val/1
  PreConitionRunnable_sys/278(StSrvCfg_Md7_Val_write) -> StSrvCfg_Md7_Val/1
  PreConitionRunnable_sys/279(StSrvCfg_Md8_Val_write) -> StSrvCfg_Md8_Val/1
  PreConitionRunnable_sys/280(StSrvCfg_Md9_Val_write) -> StSrvCfg_Md9_Val/1
  PreConitionRunnable_sys/281(VipMdLtAvl_Val_write) -> VipMdLtAvl_Val/1
  PreConitionRunnable_sys/282(VipMdRtAvl_Val_write) -> VipMdRtAvl_Val/1
  PreConitionRunnable/1 -> PreConitionRunnable_sys/Trigger
  SecRwLtStFrwdBkwdPos_Val/1 -> PreConitionRunnable_sys/54(SecRwLtStFrwdBkwdPos_Val_read)
  SecRwLtStFrwdBkwdPosV_Val/1 -> PreConitionRunnable_sys/55(SecRwLtStFrwdBkwdPosV_Val_read)
  SecRwRtStFrwdBkwdPos_Val/1 -> PreConitionRunnable_sys/56(SecRwRtStFrwdBkwdPos_Val_read)
  SecRwRtStFrwdBkwdPosV_Val/1 -> PreConitionRunnable_sys/57(SecRwRtStFrwdBkwdPosV_Val_read)
  AcsEntry4s2LPosLrnd_Val/1 -> PreConitionRunnable_sys/58(AcsEntry4s2LPosLrnd_Val_read)
  AcsEntry4s2RPosLrnd_Val/1 -> PreConitionRunnable_sys/59(AcsEntry4s2RPosLrnd_Val_read)
  AcsEntryAll4sBwdPosLrnd_Val/1 -> PreConitionRunnable_sys/60(AcsEntryAll4sBwdPosLrnd_Val_read)
  AcsEntryAll4sFwdPosLrnd_Val/1 -> PreConitionRunnable_sys/61(AcsEntryAll4sFwdPosLrnd_Val_read)
  AcsExit4s2LPosLrnd_Val/1 -> PreConitionRunnable_sys/62(AcsExit4s2LPosLrnd_Val_read)
  AcsExit4s2RPosLrnd_Val/1 -> PreConitionRunnable_sys/63(AcsExit4s2RPosLrnd_Val_read)
  PreConitionRunnable_sys/283(AcsEntry4s2LAvl_Val_write) -> AcsEntry4s2LAvl_Val/1
  PreConitionRunnable_sys/284(AcsEntry4s2RAvl_Val_write) -> AcsEntry4s2RAvl_Val/1
  PreConitionRunnable_sys/285(AcsEntryAll4sBwdAvl_Val_write) -> AcsEntryAll4sBwdAvl_Val/1
  PreConitionRunnable_sys/286(AcsEntryAll4sFwdAvl_Val_write) -> AcsEntryAll4sFwdAvl_Val/1
  PreConitionRunnable_sys/287(AcsExit4s2LAvl_Val_write) -> AcsExit4s2LAvl_Val/1
  PreConitionRunnable_sys/288(AcsExit4s2RAvl_Val_write) -> AcsExit4s2RAvl_Val/1
  IfVeSMSbPassReclinerPosLrnd_Val/1 -> PreConitionRunnable_sys/64(IfVeSMSbPassReclinerPosLrnd_Val_read)
  IfVeSMSbunfold3LPosLrnd_Val/1 -> PreConitionRunnable_sys/65(IfVeSMSbunfold3LPosLrnd_Val_read)
  IfVeSMSbunfold3RPosLrnd_Val/1 -> PreConitionRunnable_sys/66(IfVeSMSbunfold3RPosLrnd_Val_read)
  NotCoDrvStOccStatBDFSrc_Val/1 -> PreConitionRunnable_sys/67(NotCoDrvStOccStatBDFSrc_Val_read)
  IfVeSMSbVIPLtOutPosLrnd_Val/1 -> PreConitionRunnable_sys/68(IfVeSMSbVIPLtOutPosLrnd_Val_read)
  IfVeSMSbVIPRtOutPosLrnd_Val/1 -> PreConitionRunnable_sys/69(IfVeSMSbVIPRtOutPosLrnd_Val_read)
  IfVeSMSuThdRwLtStCshnFldUpwdDnwdPos_Val/1 -> PreConitionRunnable_sys/70(IfVeSMSuThdRwLtStCshnFldUpwdDnwdPos_Val_read)
  IfVeSMSuThdRwLtStCshnFldUpwdDnwdPosV_Val/1 -> PreConitionRunnable_sys/71(IfVeSMSuThdRwLtStCshnFldUpwdDnwdPosV_Val_read)
  IfVeSMSuThdRwRtStCshnFldUpwdDnwdPos_Val/1 -> PreConitionRunnable_sys/72(IfVeSMSuThdRwRtStCshnFldUpwdDnwdPos_Val_read)
  IfVeSMSuThdRwRtStCshnFldUpwdDnwdPosV_Val/1 -> PreConitionRunnable_sys/73(IfVeSMSuThdRwRtStCshnFldUpwdDnwdPosV_Val_read)
  PreConitionRunnable_sys/289(PasReclinerAvl_Val_write) -> PasReclinerAvl_Val/1
  PreConitionRunnable_sys/290(unfold3LAvl_Val_write) -> unfold3LAvl_Val/1
  PreConitionRunnable_sys/291(unfold3RAvl_Val_write) -> unfold3RAvl_Val/1
  PreConitionRunnable_sys/292(VipLtOutMdAvl_Val_write) -> VipLtOutMdAvl_Val/1
  PreConitionRunnable_sys/293(VipRtOutMdAvl_Val_write) -> VipRtOutMdAvl_Val/1
  ThdRwLtStChldLkReq_Val/1 -> PreConitionRunnable_sys/74(ThdRwLtStChldLkReq_Val_read)
  NotSecRowLeStOccStatBDFSrc_Val/1 -> PreConitionRunnable_sys/75(NotSecRowLeStOccStatBDFSrc_Val_read)
  NotSecRowRtStOccStatBDFSrc_Val/1 -> PreConitionRunnable_sys/76(NotSecRowRtStOccStatBDFSrc_Val_read)
  PreConitionRunnable_sys/294(PasReclinerExitAvl_Val_write) -> PasReclinerExitAvl_Val/1
  IfVeSMSbSecRwLtStBkReclnUpwdDnwdPosV_Val/1 -> PreConitionRunnable_sys/77(IfVeSMSbSecRwLtStBkReclnUpwdDnwdPosV_Val_read)
  IfVeSMSbSecRwRtStBkReclnUpwdDnwdPosV_Val/1 -> PreConitionRunnable_sys/78(IfVeSMSbSecRwRtStBkReclnUpwdDnwdPosV_Val_read)
  IfVeSMSuSecRwLtStBkReclnUpwdDnwdPos_Val/1 -> PreConitionRunnable_sys/79(IfVeSMSuSecRwLtStBkReclnUpwdDnwdPos_Val_read)
  IfVeSMSuSecRwRtStBkReclnUpwdDnwdPos_Val/1 -> PreConitionRunnable_sys/80(IfVeSMSuSecRwRtStBkReclnUpwdDnwdPos_Val_read)
  PreConitionRunnable_sys/295(StPassCmprtMdCtrl_Md53_VCUAvl_Val_write) -> StPassCmprtMdCtrl_Md53_VCUAvl_Val/1
  PreConitionRunnable_sys/296(StPassCmprtMdCtrl_Md53_VCUCfg_Val_write) -> StPassCmprtMdCtrl_Md53_VCUCfg_Val/1
  PreConitionRunnable_sys/297(StPassCmprtMdCtrl_Md56_VCUAvl_Val_write) -> StPassCmprtMdCtrl_Md56_VCUAvl_Val/1
  PreConitionRunnable_sys/298(StPassCmprtMdCtrl_Md56_VCUCfg_Val_write) -> StPassCmprtMdCtrl_Md56_VCUCfg_Val/1
  PreConitionRunnable_sys/299(StPassCmprtMdCtrl_Md57_VCUAvl_Val_write) -> StPassCmprtMdCtrl_Md57_VCUAvl_Val/1
  PreConitionRunnable_sys/300(StPassCmprtMdCtrl_Md57_VCUCfg_Val_write) -> StPassCmprtMdCtrl_Md57_VCUCfg_Val/1
  PreConitionRunnable_sys/301(StPassCmprtMdCtrl_Md58_VCUAvl_Val_write) -> StPassCmprtMdCtrl_Md58_VCUAvl_Val/1
  PreConitionRunnable_sys/302(StPassCmprtMdCtrl_Md58_VCUCfg_Val_write) -> StPassCmprtMdCtrl_Md58_VCUCfg_Val/1
  IfVeSMSbPasReclinerPosAvail_Val/1 -> PreConitionRunnable_sys/81(IfVeSMSbPasReclinerPosAvail_Val_read)
  PreConitionRunnable_sys/303(Big4SeatAvl_Val_write) -> Big4SeatAvl_Val/1
  WholeVehMemPosLrnd_Val/1 -> PreConitionRunnable_sys/82(WholeVehMemPosLrnd_Val_read)
  PreConitionRunnable_sys/304(StPassCmprtMdCtrl_Md61_VCUAvl_Val_write) -> StPassCmprtMdCtrl_Md61_VCUAvl_Val/1
  PreConitionRunnable_sys/305(StPassCmprtMdCtrl_Md62_VCUAvl_Val_write) -> StPassCmprtMdCtrl_Md62_VCUAvl_Val/1
  Md61PassStBkReclnTrgtPos_Val/1 -> PreConitionRunnable_sys/83(Md61PassStBkReclnTrgtPos_Val_read)
  Md61ThdRwLtStCshnFldUpwdDnwdTrgtPos_Val/1 -> PreConitionRunnable_sys/84(Md61ThdRwLtStCshnFldUpwdDnwdTrgtPos_Val_read)
  Md61ThdRwRtStCshnFldUpwdDnwdTrgtPos_Val/1 -> PreConitionRunnable_sys/85(Md61ThdRwRtStCshnFldUpwdDnwdTrgtPos_Val_read)
  Md62PassStBkReclnTrgtPos_Val/1 -> PreConitionRunnable_sys/86(Md62PassStBkReclnTrgtPos_Val_read)
  Md62ThdRwLtStCshnFldUpwdDnwdTrgtPos_Val/1 -> PreConitionRunnable_sys/87(Md62ThdRwLtStCshnFldUpwdDnwdTrgtPos_Val_read)
  Md62ThdRwRtStCshnFldUpwdDnwdTrgtPos_Val/1 -> PreConitionRunnable_sys/88(Md62ThdRwRtStCshnFldUpwdDnwdTrgtPos_Val_read)
  PreConitionRunnable_sys/306(M61WholeVehMemAvl_Val_write) -> M61WholeVehMemAvl_Val/1
  PreConitionRunnable_sys/307(M62WholeVehMemAvl_Val_write) -> M62WholeVehMemAvl_Val/1
  PreConitionRunnable_sys/308(StPassCmprtMdCtrl_Md61_VCUCfg_Val_write) -> StPassCmprtMdCtrl_Md61_VCUCfg_Val/1
  PreConitionRunnable_sys/309(StPassCmprtMdCtrl_Md62_VCUCfg_Val_write) -> StPassCmprtMdCtrl_Md62_VCUCfg_Val/1
